simulink model "CRITIS_1_full"  (R2022b)
settings: Solver=VariableStepAuto  StartTime=0.0  StopTime=7  RelTol=1e-3
(part 6 of 13)

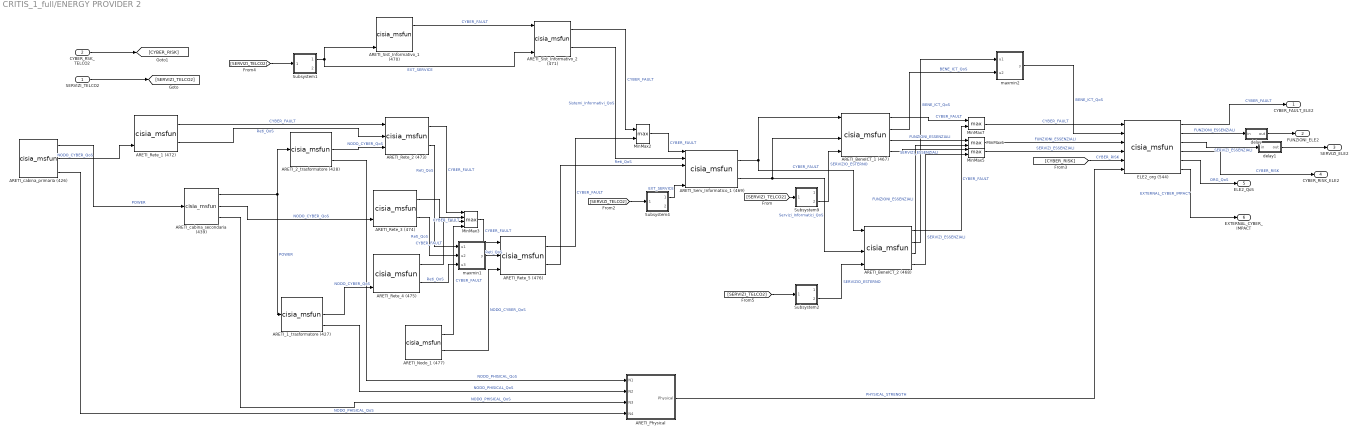
== system CRITIS_1_full/ENERGY PROVIDER 2 ==
  SERVIZI_TELCO2 : Inport
  CYBER_RSK_TELCO2 : Inport  Port=2
  ARETI_1_trasformatore (427) : M-S-Function  FunctionName=cisia_msfun  Parameters=Parameter1, Parameter2, Parameter3, resources, Parameter10, codeupdate, step_received, step_computed, dynamic_computed, step_sended, id_entity, id_project, id_type, name_type, color  mask(S-function:msfcn_unit_delay){Parameter1='ARETI_1_trasformatore', Parameter2=1, Parameter3='Iside', resources=|, Parameter10=off, codeupdate=off, step_received=|, step_computed=, dynamic_computed=, step_sended=|, id_entity=427, id_project=14, id_type=105, name_type=Nodo_Trasformatore, color=#DCF6F7}
      mask resources=|
      | *** INPUT RESOURCES ***
      | NUM_INPUTS 1
      | POWER (1)
      |
      | *** STATE VARIABLES ***
      | NUM_VARIABLES 8
      | Operative_Level(NUMERIC)(1)(1)
      | Mechanical_Fault(NUMERIC)(1)(0)
      | Power_Fault(NUMERIC)(1)(0)
      | Fire_Fault(NUMERIC)(1)(0)
      | Physical_Fault(NUMERIC)(1)(0)
      | Op_Level2(NUMERIC_ARRAY)(2)(0  0)
      | Possibility_Value(NUMERIC)(1)(0)
      | Necessity_Value(NUMERIC)(1)(0)
      |
      | *** OUTPUT RESOURCES ***
      | NUM_OUTPUTS 3
      | POWER_QoS (1)
      | NODO_CYBER_QoS (2)
      | NODO_PHISICAL_QoS (1)
      mask step_received=|
      | Power_Fault = 1-POWER;
      |
      | Physical_Fault = max([Mechanical_Fault Fire_Fault]);
      |
      | Operative_Level = (1-Power_Fault)*(1-Physical_Fault);
      |
      | % Il primo elemento rappersenta possibility e si combima
      | % con il max in quanto rende conto del caso migliore
      | % (perche OL)
      |
      | Op_Level2(1)=  min([1-Power_Fault 1-Physical_Fault]);
      |
      | % Il secondo elemento rappersenta necessity e si combima
      | % con il min in quanto rende conto del caso peggiore
      | % (perche OL)
      |
      | Op_Level2(2)= min([1-Power_Fault 1-Physical_Fault]);
      |
      | Possibility_Value = Op_Level2(1);
      | Necessity_Value = Op_Level2(2);
      mask step_sended=|
      | POWER_QoS = 1-Power_Fault;
      |
      | NODO_CYBER_QoS=Op_Level2;
      |
      | NODO_PHISICAL_QoS=1-Physical_Fault;
      mask prompts: Parameter1 "entity name"; Parameter2 "sampling time"; Parameter3 "project"; resources "input resources and state variables"; Parameter10 "Bring state variables to output"; codeupdate "update code from mask"
      mask help: This is a level-2 MATLAB file S-function which demonstrates CISIA entity
      mask DialogControl Container1 Prompt: All parameters
      mask Display: disp('Nodo_Trasformatore')
  ARETI_2_trasformatore (428) : M-S-Function  FunctionName=cisia_msfun  Parameters=Parameter1, Parameter2, Parameter3, resources, Parameter10, codeupdate, step_received, step_computed, dynamic_computed, step_sended, id_entity, id_project, id_type, name_type, color  mask(S-function:msfcn_unit_delay){Parameter1='ARETI_2_trasformatore', Parameter2=1, Parameter3='Iside', resources=|, Parameter10=off, codeupdate=off, step_received=|, step_computed=, dynamic_computed=, step_sended=|, id_entity=428, id_project=14, id_type=105, name_type=Nodo_Trasformatore, color=#DCF6F7}
      mask resources=|
      | *** INPUT RESOURCES ***
      | NUM_INPUTS 1
      | POWER (1)
      |
      | *** STATE VARIABLES ***
      | NUM_VARIABLES 8
      | Operative_Level(NUMERIC)(1)(1)
      | Mechanical_Fault(NUMERIC)(1)(0)
      | Power_Fault(NUMERIC)(1)(0)
      | Fire_Fault(NUMERIC)(1)(0)
      | Physical_Fault(NUMERIC)(1)(0)
      | Op_Level2(NUMERIC_ARRAY)(2)(0  0)
      | Possibility_Value(NUMERIC)(1)(0)
      | Necessity_Value(NUMERIC)(1)(0)
      |
      | *** OUTPUT RESOURCES ***
      | NUM_OUTPUTS 3
      | POWER_QoS (1)
      | NODO_CYBER_QoS (2)
      | NODO_PHISICAL_QoS (1)
      mask step_received=|
      | Power_Fault = 1-POWER;
      |
      | Physical_Fault = max([Mechanical_Fault Fire_Fault]);
      |
      | Operative_Level = (1-Power_Fault)*(1-Physical_Fault);
      |
      | % Il primo elemento rappersenta possibility e si combima
      | % con il max in quanto rende conto del caso migliore
      | % (perche OL)
      |
      | Op_Level2(1)=  min([1-Power_Fault 1-Physical_Fault]);
      |
      | % Il secondo elemento rappersenta necessity e si combima
      | % con il min in quanto rende conto del caso peggiore
      | % (perche OL)
      |
      | Op_Level2(2)= min([1-Power_Fault 1-Physical_Fault]);
      |
      | Possibility_Value = Op_Level2(1);
      | Necessity_Value = Op_Level2(2);
      mask step_sended=|
      | POWER_QoS = 1-Power_Fault;
      |
      | NODO_CYBER_QoS=Op_Level2;
      |
      | NODO_PHISICAL_QoS=1-Physical_Fault;
      mask prompts: Parameter1 "entity name"; Parameter2 "sampling time"; Parameter3 "project"; resources "input resources and state variables"; Parameter10 "Bring state variables to output"; codeupdate "update code from mask"
      mask help: This is a level-2 MATLAB file S-function which demonstrates CISIA entity
      mask DialogControl Container1 Prompt: All parameters
      mask Display: disp('Nodo_Trasformatore')
  ARETI_BeneICT_1 (467) : M-S-Function  FunctionName=cisia_msfun  Parameters=Parameter1, Parameter2, Parameter3, resources, Parameter10, codeupdate, step_received, step_computed, dynamic_computed, step_sended, id_entity, id_project, id_type, name_type, color  mask(S-function:msfcn_unit_delay){Parameter1='ARETI_BeneICT_1', Parameter2=1, Parameter3='Iside', resources=|, Parameter10=off, codeupdate=off, step_received=|, step_computed=, dynamic_computed=, step_sended=|, id_entity=467, id_project=14, id_type=108, name_type=BeneICT, color=#64D413}
      mask resources=|
      | *** INPUT RESOURCES ***
      | NUM_INPUTS 6
      | CYBER_FAULT (25)
      | Sistemi_Informativi_QoS (2)
      | Reti_QoS (2)
      | Servizi_Informatici_QoS (2)
      | BENE_ICT_QoS (2)
      | SERVIZIO_ESTERNO (20)
      |
      | *** STATE VARIABLES ***
      | NUM_VARIABLES 34
      | Operative_Level(NUMERIC)(1)(1)
      | Dos_attack(NUMERIC)(1)(0)
      | MITM_attack(NUMERIC)(1)(0)
      | Virus_Attack(NUMERIC)(1)(0)
      | Port_Scan_Attack(NUMERIC)(1)(0)
      | Cyber_Fault(NUMERIC_ARRAY)(25)(0  0  0  0  0  0  0  0  0  0  0  0  0  0  0  0  0  0  0  0  0  0  0  0  0)
      | BGP_hijacking(NUMERIC)(1)(0)
      | Unauthorized_Access(NUMERIC)(1)(0)
      | Consumed_Services(NUMERIC_ARRAY)(10)(0  0  0  0  0  0  0  0  0  0)
      | Service_Fault(NUMERIC)(1)(0)
      | BotNet_Attack(NUMERIC)(1)(0)
      | Data_Corruption(NUMERIC)(1)(0)
      | Rouge_Access(NUMERIC)(1)(0)
      | syslog_adm_login(NUMERIC)(1)(0)
      | SW_Change(NUMERIC)(1)(0)
      | Config_Change(NUMERIC)(1)(0)
      | Port_Saturation(NUMERIC)(1)(0)
      | Congestion_Fault(NUMERIC)(1)(0)
      | Route_Poisoning(NUMERIC)(1)(0)
      | Interface_Down(NUMERIC)(1)(0)
      | Port_Isolation(NUMERIC)(1)(0)
      | Unknown_Device(NUMERIC)(1)(0)
      | USB_Device_Insertion(NUMERIC)(1)(0)
      | SW_Fault(NUMERIC)(1)(0)
      | Servizi_Essenziali(NUMERIC_ARRAY)(10)(1  0  0  0  0  0  0  0  0  0)
      | Funzioni_Essenziali(NUMERIC_ARRAY)(10)(0  0  0  0  0  0  0  0  0  0)
      | Consumed_Functions(NUMERIC_ARRAY)(10)(0  0  0  0  0  0  0  0  0  0)
      | Internal_Cyber_Risk(NUMERIC)(1)(0)
      | Data_Breach(NUMERIC)(1)(0)
      | availability_fault(NUMERIC)(1)(0)
      | Ransomware(NUMERIC)(1)(0)
      | Op_Level2(NUMERIC_ARRAY)(2)(0  0)
      | Possibility_Value(NUMERIC)(1)(0)
      | Necessity_Value(NUMERIC)(1)(0)
      |
      | *** OUTPUT RESOURCES ***
      | NUM_OUTPUTS 4
      | CYBER_FAULT (25)
      | BENE_ICT_QoS (2)
      | FUNZIONI_ESSENZIALI (10)
      | SERVIZI_ESSENZIALI (10)
      mask step_received=|
      | cyber_event=zeros(1,25);
      | cyber_event(1)=Dos_attack;
      | cyber_event(2)=MITM_attack;
      | cyber_event(3)=Virus_Attack;
      | cyber_event(4)=Port_Scan_Attack;
      | cyber_event(5)=BGP_hijacking;
      | cyber_event(6)=BotNet_Attack;
      | cyber_event(7)=Data_Corruption;
      | cyber_event(8)=SW_Change;
      | cyber_event(9)=Config_Change;
      | cyber_event(10)=Port_Saturation;
      | cyber_event(11)=Data_Breach;
      | cyber_event(12)=Unauthorized_Access;
      | cyber_event(13)=Unknown_Device;
      | cyber_event(14)=Congestion_Fault;
      | cyber_event(15)=Interface_Down;
      | cyber_event(16)=Port_Isolation;
      | cyber_event(17)=Rouge_Access;
      | cyber_event(18)=Route_Poisoning;
      | cyber_event(19)=SW_Fault;
      | cyber_event(20)=syslog_adm_login;
      | cyber_event(21)=USB_Device_Insertion;
      | cyber_event(22)=Ransomware;
      | cyber_event(23)=0;
      | cyber_event(24)=0;
      | cyber_event(25)=0;
      |
      | Cyber_Fault=max(CYBER_FAULT, transpose(cyber_event));
      |
      | Consumed_Services=SERVIZIO_ESTERNO(1:10);
      | Consumed_Functions=SERVIZIO_ESTERNO(11:20);
      |
      | Service_Fault=max(abs(Servizi_Essenziali-Consumed_Services));
      |
      | availability_fault=1-min([(1-0.5*max(Cyber_Fault)) min(Reti_QoS) min(Sistemi_Informativi_QoS) min(Servizi_Informatici_QoS) min(BENE_ICT_QoS)]);
      |
      | Operative_Level=min([(1-0.5*max(Cyber_Fault)) mean(Reti_QoS) mean(Sistemi_Informativi_QoS) mean(Servizi_Informatici_QoS) mean(BENE_ICT_QoS) 1-Service_Fault]);
      |
      | % Il primo elemento rappersenta possibility e si combima
      | % con il max in quanto rende conto del caso migliore
      | % (perche OL)
      |
      | BNICT=BENE_ICT_QoS;
      |
      | Op_Level2(1)=  min([1-0.3*max(Cyber_Fault) max([use_elem(Reti_QoS,1) use_elem(Sistemi_Informativi_QoS,1) use_elem(Servizi_Informatici_QoS,1) use_elem(BENE_ICT_QoS,1)]) 1-Service_Fault]);
      |
      | % Il secondo elemento rappresenta necessity e si combima
      | % con il min in quanto rende conto del caso peggiore
      | % (perche OL)
      |
      |
      |
      | Op_Level2(2)= min([1-0.6*max(Cyber_Fault) min([use_elem(Reti_QoS,2) use_elem(Sistemi_Informativi_QoS,2) use_elem(Servizi_Informatici_QoS,2) use_elem(BENE_ICT_QoS,2)]) 1-Service_Fault]);
      |
      | Possibility_Value = Op_Level2(1);
      | Necessity_Value = Op_Level2(2);
      mask step_sended=|
      | CYBER_FAULT=Cyber_Fault;
      |
      | FUNZIONI_ESSENZIALI=(1-availability_fault)*Funzioni_Essenziali.*Consumed_Functions;
      |
      | SERVIZI_ESSENZIALI=(1-availability_fault)*Servizi_Essenziali.*Consumed_Services;
      |
      | BENE_ICT_QoS=Op_Level2;
      mask prompts: Parameter1 "entity name"; Parameter2 "sampling time"; Parameter3 "project"; resources "input resources and state variables"; Parameter10 "Bring state variables to output"; codeupdate "update code from mask"
      mask help: This is a level-2 MATLAB file S-function which demonstrates CISIA entity
      mask DialogControl Container1 Prompt: All parameters
      mask Display: disp('BeneICT');port_label('input',2,'\color{yellow}\spadesuit','texmode','on');port_label('input',3,'\color{yellow}\spadesuit','texmode','on');port_label('input',5,'\color{yellow}\spadesuit','texmode','on')
  ARETI_BeneICT_2 (468) : M-S-Function  FunctionName=cisia_msfun  Parameters=Parameter1, Parameter2, Parameter3, resources, Parameter10, codeupdate, step_received, step_computed, dynamic_computed, step_sended, id_entity, id_project, id_type, name_type, color  mask(S-function:msfcn_unit_delay){Parameter1='ARETI_BeneICT_2', Parameter2=1, Parameter3='Iside', resources=|, Parameter10=off, codeupdate=off, step_received=|, step_computed=, dynamic_computed=, step_sended=|, id_entity=468, id_project=14, id_type=108, name_type=BeneICT, color=#64D413}
      mask resources=|
      | *** INPUT RESOURCES ***
      | NUM_INPUTS 6
      | CYBER_FAULT (25)
      | Sistemi_Informativi_QoS (2)
      | Reti_QoS (2)
      | Servizi_Informatici_QoS (2)
      | BENE_ICT_QoS (2)
      | SERVIZIO_ESTERNO (20)
      |
      | *** STATE VARIABLES ***
      | NUM_VARIABLES 34
      | Operative_Level(NUMERIC)(1)(1)
      | Dos_attack(NUMERIC)(1)(0)
      | MITM_attack(NUMERIC)(1)(0)
      | Virus_Attack(NUMERIC)(1)(0)
      | Port_Scan_Attack(NUMERIC)(1)(0)
      | Cyber_Fault(NUMERIC_ARRAY)(25)(0  0  0  0  0  0  0  0  0  0  0  0  0  0  0  0  0  0  0  0  0  0  0  0  0)
      | BGP_hijacking(NUMERIC)(1)(0)
      | Unauthorized_Access(NUMERIC)(1)(0)
      | Consumed_Services(NUMERIC_ARRAY)(10)(0  0  0  0  0  0  0  0  0  0)
      | Service_Fault(NUMERIC)(1)(0)
      | BotNet_Attack(NUMERIC)(1)(0)
      | Data_Corruption(NUMERIC)(1)(0)
      | Rouge_Access(NUMERIC)(1)(0)
      | syslog_adm_login(NUMERIC)(1)(0)
      | SW_Change(NUMERIC)(1)(0)
      | Config_Change(NUMERIC)(1)(0)
      | Port_Saturation(NUMERIC)(1)(0)
      | Congestion_Fault(NUMERIC)(1)(0)
      | Route_Poisoning(NUMERIC)(1)(0)
      | Interface_Down(NUMERIC)(1)(0)
      | Port_Isolation(NUMERIC)(1)(0)
      | Unknown_Device(NUMERIC)(1)(0)
      | USB_Device_Insertion(NUMERIC)(1)(0)
      | SW_Fault(NUMERIC)(1)(0)
      | Servizi_Essenziali(NUMERIC_ARRAY)(10)(0  1  0  0  0  0  0  0  0  0)
      | Funzioni_Essenziali(NUMERIC_ARRAY)(10)(0  0  0  0  0  0  0  0  0  0)
      | Consumed_Functions(NUMERIC_ARRAY)(10)(0  0  0  0  0  0  0  0  0  0)
      | Internal_Cyber_Risk(NUMERIC)(1)(0)
      | Data_Breach(NUMERIC)(1)(0)
      | availability_fault(NUMERIC)(1)(0)
      | Ransomware(NUMERIC)(1)(0)
      | Op_Level2(NUMERIC_ARRAY)(2)(0  0)
      | Possibility_Value(NUMERIC)(1)(0)
      | Necessity_Value(NUMERIC)(1)(0)
      |
      | *** OUTPUT RESOURCES ***
      | NUM_OUTPUTS 4
      | CYBER_FAULT (25)
      | BENE_ICT_QoS (2)
      | FUNZIONI_ESSENZIALI (10)
      | SERVIZI_ESSENZIALI (10)
      mask step_received=|
      | cyber_event=zeros(1,25);
      | cyber_event(1)=Dos_attack;
      | cyber_event(2)=MITM_attack;
      | cyber_event(3)=Virus_Attack;
      | cyber_event(4)=Port_Scan_Attack;
      | cyber_event(5)=BGP_hijacking;
      | cyber_event(6)=BotNet_Attack;
      | cyber_event(7)=Data_Corruption;
      | cyber_event(8)=SW_Change;
      | cyber_event(9)=Config_Change;
      | cyber_event(10)=Port_Saturation;
      | cyber_event(11)=Data_Breach;
      | cyber_event(12)=Unauthorized_Access;
      | cyber_event(13)=Unknown_Device;
      | cyber_event(14)=Congestion_Fault;
      | cyber_event(15)=Interface_Down;
      | cyber_event(16)=Port_Isolation;
      | cyber_event(17)=Rouge_Access;
      | cyber_event(18)=Route_Poisoning;
      | cyber_event(19)=SW_Fault;
      | cyber_event(20)=syslog_adm_login;
      | cyber_event(21)=USB_Device_Insertion;
      | cyber_event(22)=Ransomware;
      | cyber_event(23)=0;
      | cyber_event(24)=0;
      | cyber_event(25)=0;
      |
      | Cyber_Fault=max(CYBER_FAULT, transpose(cyber_event));
      |
      | Consumed_Services=SERVIZIO_ESTERNO(1:10);
      | Consumed_Functions=SERVIZIO_ESTERNO(11:20);
      |
      | Service_Fault=max(abs(Servizi_Essenziali-Consumed_Services));
      |
      | availability_fault=1-min([(1-0.5*max(Cyber_Fault)) min(Reti_QoS) min(Sistemi_Informativi_QoS) min(Servizi_Informatici_QoS) min(BENE_ICT_QoS)]);
      |
      | Operative_Level=min([(1-0.5*max(Cyber_Fault)) mean(Reti_QoS) mean(Sistemi_Informativi_QoS) mean(Servizi_Informatici_QoS) mean(BENE_ICT_QoS) 1-Service_Fault]);
      |
      | % Il primo elemento rappersenta possibility e si combima
      | % con il max in quanto rende conto del caso migliore
      | % (perche OL)
      |
      | BNICT=BENE_ICT_QoS;
      |
      | Op_Level2(1)=  min([1-0.3*max(Cyber_Fault) max([use_elem(Reti_QoS,1) use_elem(Sistemi_Informativi_QoS,1) use_elem(Servizi_Informatici_QoS,1) use_elem(BENE_ICT_QoS,1)]) 1-Service_Fault]);
      |
      | % Il secondo elemento rappresenta necessity e si combima
      | % con il min in quanto rende conto del caso peggiore
      | % (perche OL)
      |
      |
      |
      | Op_Level2(2)= min([1-0.6*max(Cyber_Fault) min([use_elem(Reti_QoS,2) use_elem(Sistemi_Informativi_QoS,2) use_elem(Servizi_Informatici_QoS,2) use_elem(BENE_ICT_QoS,2)]) 1-Service_Fault]);
      |
      | Possibility_Value = Op_Level2(1);
      | Necessity_Value = Op_Level2(2);
      mask step_sended=|
      | CYBER_FAULT=Cyber_Fault;
      |
      | FUNZIONI_ESSENZIALI=(1-availability_fault)*Funzioni_Essenziali.*Consumed_Functions;
      |
      | SERVIZI_ESSENZIALI=(1-availability_fault)*Servizi_Essenziali.*Consumed_Services;
      |
      | BENE_ICT_QoS=Op_Level2;
      mask prompts: Parameter1 "entity name"; Parameter2 "sampling time"; Parameter3 "project"; resources "input resources and state variables"; Parameter10 "Bring state variables to output"; codeupdate "update code from mask"
      mask help: This is a level-2 MATLAB file S-function which demonstrates CISIA entity
      mask DialogControl Container1 Prompt: All parameters
      mask Display: disp('BeneICT');port_label('input',2,'\color{yellow}\spadesuit','texmode','on');port_label('input',3,'\color{yellow}\spadesuit','texmode','on');port_label('input',5,'\color{yellow}\spadesuit','texmode','on')
  ARETI_Nodo_1 (477) : M-S-Function  FunctionName=cisia_msfun  Parameters=Parameter1, Parameter2, Parameter3, resources, Parameter10, codeupdate, step_received, step_computed, dynamic_computed, step_sended, id_entity, id_project, id_type, name_type, color  mask(S-function:msfcn_unit_delay){Parameter1='ARETI_Nodo_1', Parameter2=1, Parameter3='Iside', resources=|, Parameter10=off, codeupdate=off, step_received=|, step_computed=, dynamic_computed=, step_sended=|, id_entity=477, id_project=14, id_type=109, name_type=Nodo_Datacenter, color=#DCF6F7}
      mask resources=|
      | *** INPUT RESOURCES ***
      | NUM_INPUTS 0
      |
      | *** STATE VARIABLES ***
      | NUM_VARIABLES 32
      | Operative_Level(NUMERIC)(1)(1)
      | Dos_attack(NUMERIC)(1)(0)
      | MITM_attack(NUMERIC)(1)(0)
      | Virus_Attack(NUMERIC)(1)(0)
      | Port_Scan_Attack(NUMERIC)(1)(0)
      | Cyber_Fault(NUMERIC_ARRAY)(25)(0  0  0  0  0  0  0  0  0  0  0  0  0  0  0  0  0  0  0  0  0  0  0  0  0)
      | BGP_hijacking(NUMERIC)(1)(0)
      | Mechanical_Fault(NUMERIC)(1)(0)
      | Unauthorized_Access(NUMERIC)(1)(0)
      | Conn_Fault(NUMERIC)(1)(0)
      | BotNet_Attack(NUMERIC)(1)(0)
      | Data_Corruption(NUMERIC)(1)(0)
      | Rouge_Access(NUMERIC)(1)(0)
      | syslog_adm_login(NUMERIC)(1)(0)
      | SW_Change(NUMERIC)(1)(0)
      | Config_Change(NUMERIC)(1)(0)
      | Port_Saturation(NUMERIC)(1)(0)
      | Congestion_Fault(NUMERIC)(1)(0)
      | Route2(NUMERIC)(1)(0)
      | Route_Poisoning(NUMERIC)(1)(0)
      | Interface_Down(NUMERIC)(1)(0)
      | Port_Isolation(NUMERIC)(1)(0)
      | Unknown_Device(NUMERIC)(1)(0)
      | USB_Device_Insertion(NUMERIC)(1)(0)
      | GEO_localization(STRING)(100)()
      | SW_Fault(NUMERIC)(1)(0)
      | Internal_Cyber_Risk(NUMERIC)(1)(0)
      | Data_Breach(NUMERIC)(1)(0)
      | Ransomware(NUMERIC)(1)(0)
      | Op_Level2(NUMERIC_ARRAY)(2)(0  0)
      | Possibility_Value(NUMERIC)(1)(0)
      | Necessity_Value(NUMERIC)(1)(0)
      |
      | *** OUTPUT RESOURCES ***
      | NUM_OUTPUTS 2
      | CYBER_FAULT (25)
      | NODO_CYBER_QoS (2)
      mask step_received=|
      | cyber_event=zeros(1,25);
      | cyber_event(1)=Dos_attack;
      | cyber_event(2)=MITM_attack;
      | cyber_event(3)=Virus_Attack;
      | cyber_event(4)=Port_Scan_Attack;
      | cyber_event(5)=BGP_hijacking;
      | cyber_event(6)=BotNet_Attack;
      | cyber_event(7)=Data_Corruption;
      | cyber_event(8)=SW_Change;
      | cyber_event(9)=Config_Change;
      | cyber_event(10)=Port_Saturation;
      | cyber_event(11)=Data_Breach;
      | cyber_event(12)=Unauthorized_Access;
      | cyber_event(13)=Unknown_Device;
      | cyber_event(14)=Congestion_Fault;
      | cyber_event(15)=Interface_Down;
      | cyber_event(16)=Port_Isolation;
      | cyber_event(17)=Rouge_Access;
      | cyber_event(18)=Route_Poisoning;
      | cyber_event(19)=SW_Fault;
      | cyber_event(20)=syslog_adm_login;
      | cyber_event(21)=USB_Device_Insertion;
      | cyber_event(22)=Ransomware;
      | cyber_event(23)=0;
      | cyber_event(24)=0;
      | cyber_event(25)=0;
      |
      | Cyber_Fault=transpose(cyber_event);
      |
      | Conn_Fault=max([Dos_attack BGP_hijacking Route_Poisoning Interface_Down Mechanical_Fault] );
      |
      |
      | Operative_Level=min((1-Conn_Fault),(1-0.5*max(Cyber_Fault)));
      |
      | % Il primo elemento rappersenta possibility e si combima
      | % con il max in quanto rende conto del caso migliore
      | % (perche OL)
      |
      | Op_Level2(1)=  min([1-0.3*max(Cyber_Fault) 1-Conn_Fault]);
      |
      | % Il secondo elemento rappersenta necessity e si combima
      | % con il min in quanto rende conto del caso peggiore
      | % (perche OL)
      |
      | Op_Level2(2)= min([1-0.6*max(Cyber_Fault) 1-Conn_Fault]);
      |
      | Possibility_Value = Op_Level2(1);
      | Necessity_Value = Op_Level2(2);
      mask step_sended=|
      | CYBER_FAULT=Cyber_Fault;
      |
      |
      | NODO_CYBER_QoS=Op_Level2;
      mask prompts: Parameter1 "entity name"; Parameter2 "sampling time"; Parameter3 "project"; resources "input resources and state variables"; Parameter10 "Bring state variables to output"; codeupdate "update code from mask"
      mask help: This is a level-2 MATLAB file S-function which demonstrates CISIA entity
      mask DialogControl Container1 Prompt: All parameters
      mask Display: disp('Nodo_Datacenter')
  ARETI_Physical : MATLAB Function  TreatAsAtomicUnit=on
  ARETI_Rete_1 (472) : M-S-Function  FunctionName=cisia_msfun  Parameters=Parameter1, Parameter2, Parameter3, resources, Parameter10, codeupdate, step_received, step_computed, dynamic_computed, step_sended, id_entity, id_project, id_type, name_type, color  mask(S-function:msfcn_unit_delay){Parameter1='ARETI_Rete_1', Parameter2=1, Parameter3='Iside', resources=|, Parameter10=off, codeupdate=off, step_received=|, step_computed=, dynamic_computed=, step_sended=|, id_entity=472, id_project=14, id_type=82, name_type=Reti_Sito, color=#45B5ED}
      mask resources=|
      | *** INPUT RESOURCES ***
      | NUM_INPUTS 3
      | CYBER_FAULT (25)
      | Reti_QoS (2)
      | NODO_CYBER_QoS (2)
      |
      | *** STATE VARIABLES ***
      | NUM_VARIABLES 34
      | Operative_Level(NUMERIC)(1)(1)
      | Dos_attack(NUMERIC)(1)(0)
      | MITM_attack(NUMERIC)(1)(0)
      | Virus_Attack(NUMERIC)(1)(0)
      | Port_Scan_Attack(NUMERIC)(1)(0)
      | Cyber_Fault(NUMERIC_ARRAY)(25)(0  0  0  0  0  0  0  0  0  0  0  0  0  0  0  0  0  0  0  0  0  0  0  0  0)
      | BGP_hijacking(NUMERIC)(1)(0)
      | Mechanical_Fault(NUMERIC)(1)(0)
      | Unauthorized_Access(NUMERIC)(1)(0)
      | Conn_Fault(NUMERIC)(1)(0)
      | BotNet_Attack(NUMERIC)(1)(0)
      | Data_Corruption(NUMERIC)(1)(0)
      | Rouge_Access(NUMERIC)(1)(0)
      | syslog_adm_login(NUMERIC)(1)(0)
      | SW_Change(NUMERIC)(1)(0)
      | Config_Change(NUMERIC)(1)(0)
      | Port_Saturation(NUMERIC)(1)(0)
      | Congestion_Fault(NUMERIC)(1)(0)
      | Physical_Fault(NUMERIC)(1)(0)
      | Route2(NUMERIC)(1)(0)
      | Route_Poisoning(NUMERIC)(1)(0)
      | Interface_Down(NUMERIC)(1)(0)
      | Port_Isolation(NUMERIC)(1)(0)
      | Unknown_Device(NUMERIC)(1)(0)
      | USB_Device_Insertion(NUMERIC)(1)(0)
      | Risorsa(NUMERIC)(1)(0)
      | GEO_localization(STRING)(100)()
      | SW_Fault(NUMERIC)(1)(0)
      | Internal_Cyber_Risk(NUMERIC)(1)(0)
      | Data_Breach(NUMERIC)(1)(0)
      | Ransomware(NUMERIC)(1)(0)
      | Op_Level2(NUMERIC_ARRAY)(2)(0  0)
      | Possibility_Value(NUMERIC)(1)(0)
      | Necessity_Value(NUMERIC)(1)(0)
      |
      | *** OUTPUT RESOURCES ***
      | NUM_OUTPUTS 2
      | CYBER_FAULT (25)
      | Reti_QoS (2)
      mask step_received=|
      | cyber_event=zeros(1,25);
      | cyber_event(1)=Dos_attack;
      | cyber_event(2)=MITM_attack;
      | cyber_event(3)=Virus_Attack;
      | cyber_event(4)=Port_Scan_Attack;
      | cyber_event(5)=BGP_hijacking;
      | cyber_event(6)=BotNet_Attack;
      | cyber_event(7)=Data_Corruption;
      | cyber_event(8)=SW_Change;
      | cyber_event(9)=Config_Change;
      | cyber_event(10)=Port_Saturation;
      | cyber_event(11)=Data_Breach;
      | cyber_event(12)=Unauthorized_Access;
      | cyber_event(13)=Unknown_Device;
      | cyber_event(14)=Congestion_Fault;
      | cyber_event(15)=Interface_Down;
      | cyber_event(16)=Port_Isolation;
      | cyber_event(17)=Rouge_Access;
      | cyber_event(18)=Route_Poisoning;
      | cyber_event(19)=SW_Fault;
      | cyber_event(20)=syslog_adm_login;
      | cyber_event(21)=USB_Device_Insertion;
      | cyber_event(22)=Ransomware;
      | cyber_event(23)=0;
      | cyber_event(24)=0;
      | cyber_event(25)=0;
      |
      | Cyber_Fault=max(CYBER_FAULT, transpose(cyber_event));
      |
      | Conn_Fault=max([Dos_attack BGP_hijacking Route_Poisoning Interface_Down Mechanical_Fault] );
      |
      | Operative_Level=min([(1-Conn_Fault) (1-0.5*max(Cyber_Fault))  mean(Reti_QoS)  mean(NODO_CYBER_QoS)]);
      |
      | % Il primo elemento rappersenta possibility e si combima
      | % con il max in quanto rende conto del caso migliore
      | % (perche OL)
      |
      | Op_Level2(1)=  min([1-0.3*max(Cyber_Fault) max([use_elem(Reti_QoS,1) use_elem(NODO_CYBER_QoS,1)]) 1-Conn_Fault]);
      |
      | % Il secondo elemento rappersenta necessity e si combima
      | % con il min in quanto rende conto del caso peggiore
      | % (perche OL)
      |
      | Op_Level2(2)= min([1-0.6*max(Cyber_Fault) min([use_elem(Reti_QoS,2) use_elem(NODO_CYBER_QoS,2)]) 1-Conn_Fault]);
      |
      | Possibility_Value = Op_Level2(1);
      | Necessity_Value = Op_Level2(2);
      mask step_sended=|
      | CYBER_FAULT=Cyber_Fault;
      |
      |
      | Reti_QoS=Op_Level2;
      mask prompts: Parameter1 "entity name"; Parameter2 "sampling time"; Parameter3 "project"; resources "input resources and state variables"; Parameter10 "Bring state variables to output"; codeupdate "update code from mask"
      mask help: This is a level-2 MATLAB file S-function which demonstrates CISIA entity
      mask DialogControl Container1 Prompt: All parameters
      mask Display: disp('Reti_Sito');port_label('input',1,'\color{yellow}\spadesuit','texmode','on');port_label('input',2,'\color{yellow}\spadesuit','texmode','on')
  ARETI_Rete_2 (473) : M-S-Function  FunctionName=cisia_msfun  Parameters=Parameter1, Parameter2, Parameter3, resources, Parameter10, codeupdate, step_received, step_computed, dynamic_computed, step_sended, id_entity, id_project, id_type, name_type, color  mask(S-function:msfcn_unit_delay){Parameter1='ARETI_Rete_2', Parameter2=1, Parameter3='Iside', resources=|, Parameter10=off, codeupdate=off, step_received=|, step_computed=, dynamic_computed=, step_sended=|, id_entity=473, id_project=14, id_type=82, name_type=Reti_Sito, color=#45B5ED}
      mask resources=|
      | *** INPUT RESOURCES ***
      | NUM_INPUTS 3
      | CYBER_FAULT (25)
      | Reti_QoS (2)
      | NODO_CYBER_QoS (2)
      |
      | *** STATE VARIABLES ***
      | NUM_VARIABLES 34
      | Operative_Level(NUMERIC)(1)(1)
      | Dos_attack(NUMERIC)(1)(0)
      | MITM_attack(NUMERIC)(1)(0)
      | Virus_Attack(NUMERIC)(1)(0)
      | Port_Scan_Attack(NUMERIC)(1)(0)
      | Cyber_Fault(NUMERIC_ARRAY)(25)(0  0  0  0  0  0  0  0  0  0  0  0  0  0  0  0  0  0  0  0  0  0  0  0  0)
      | BGP_hijacking(NUMERIC)(1)(0)
      | Mechanical_Fault(NUMERIC)(1)(0)
      | Unauthorized_Access(NUMERIC)(1)(0)
      | Conn_Fault(NUMERIC)(1)(0)
      | BotNet_Attack(NUMERIC)(1)(0)
      | Data_Corruption(NUMERIC)(1)(0)
      | Rouge_Access(NUMERIC)(1)(0)
      | syslog_adm_login(NUMERIC)(1)(0)
      | SW_Change(NUMERIC)(1)(0)
      | Config_Change(NUMERIC)(1)(0)
      | Port_Saturation(NUMERIC)(1)(0)
      | Congestion_Fault(NUMERIC)(1)(0)
      | Physical_Fault(NUMERIC)(1)(0)
      | Route2(NUMERIC)(1)(0)
      | Route_Poisoning(NUMERIC)(1)(0)
      | Interface_Down(NUMERIC)(1)(0)
      | Port_Isolation(NUMERIC)(1)(0)
      | Unknown_Device(NUMERIC)(1)(0)
      | USB_Device_Insertion(NUMERIC)(1)(0)
      | Risorsa(NUMERIC)(1)(0)
      | GEO_localization(STRING)(100)()
      | SW_Fault(NUMERIC)(1)(0)
      | Internal_Cyber_Risk(NUMERIC)(1)(0)
      | Data_Breach(NUMERIC)(1)(0)
      | Ransomware(NUMERIC)(1)(0)
      | Op_Level2(NUMERIC_ARRAY)(2)(0  0)
      | Possibility_Value(NUMERIC)(1)(0)
      | Necessity_Value(NUMERIC)(1)(0)
      |
      | *** OUTPUT RESOURCES ***
      | NUM_OUTPUTS 2
      | CYBER_FAULT (25)
      | Reti_QoS (2)
      mask step_received=|
      | cyber_event=zeros(1,25);
      | cyber_event(1)=Dos_attack;
      | cyber_event(2)=MITM_attack;
      | cyber_event(3)=Virus_Attack;
      | cyber_event(4)=Port_Scan_Attack;
      | cyber_event(5)=BGP_hijacking;
      | cyber_event(6)=BotNet_Attack;
      | cyber_event(7)=Data_Corruption;
      | cyber_event(8)=SW_Change;
      | cyber_event(9)=Config_Change;
      | cyber_event(10)=Port_Saturation;
      | cyber_event(11)=Data_Breach;
      | cyber_event(12)=Unauthorized_Access;
      | cyber_event(13)=Unknown_Device;
      | cyber_event(14)=Congestion_Fault;
      | cyber_event(15)=Interface_Down;
      | cyber_event(16)=Port_Isolation;
      | cyber_event(17)=Rouge_Access;
      | cyber_event(18)=Route_Poisoning;
      | cyber_event(19)=SW_Fault;
      | cyber_event(20)=syslog_adm_login;
      | cyber_event(21)=USB_Device_Insertion;
      | cyber_event(22)=Ransomware;
      | cyber_event(23)=0;
      | cyber_event(24)=0;
      | cyber_event(25)=0;
      |
      | Cyber_Fault=max(CYBER_FAULT, transpose(cyber_event));
      |
      | Conn_Fault=max([Dos_attack BGP_hijacking Route_Poisoning Interface_Down Mechanical_Fault] );
      |
      | Operative_Level=min([(1-Conn_Fault) (1-0.5*max(Cyber_Fault))  mean(Reti_QoS)  mean(NODO_CYBER_QoS)]);
      |
      | % Il primo elemento rappersenta possibility e si combima
      | % con il max in quanto rende conto del caso migliore
      | % (perche OL)
      |
      | Op_Level2(1)=  min([1-0.3*max(Cyber_Fault) max([use_elem(Reti_QoS,1) use_elem(NODO_CYBER_QoS,1)]) 1-Conn_Fault]);
      |
      | % Il secondo elemento rappersenta necessity e si combima
      | % con il min in quanto rende conto del caso peggiore
      | % (perche OL)
      |
      | Op_Level2(2)= min([1-0.6*max(Cyber_Fault) min([use_elem(Reti_QoS,2) use_elem(NODO_CYBER_QoS,2)]) 1-Conn_Fault]);
      |
      | Possibility_Value = Op_Level2(1);
      | Necessity_Value = Op_Level2(2);
      mask step_sended=|
      | CYBER_FAULT=Cyber_Fault;
      |
      |
      | Reti_QoS=Op_Level2;
      mask prompts: Parameter1 "entity name"; Parameter2 "sampling time"; Parameter3 "project"; resources "input resources and state variables"; Parameter10 "Bring state variables to output"; codeupdate "update code from mask"
      mask help: This is a level-2 MATLAB file S-function which demonstrates CISIA entity
      mask DialogControl Container1 Prompt: All parameters
      mask Display: disp('Reti_Sito')
  ARETI_Rete_3 (474) : M-S-Function  FunctionName=cisia_msfun  Parameters=Parameter1, Parameter2, Parameter3, resources, Parameter10, codeupdate, step_received, step_computed, dynamic_computed, step_sended, id_entity, id_project, id_type, name_type, color  mask(S-function:msfcn_unit_delay){Parameter1='ARETI_Rete_3', Parameter2=1, Parameter3='Iside', resources=|, Parameter10=off, codeupdate=off, step_received=|, step_computed=, dynamic_computed=, step_sended=|, id_entity=474, id_project=14, id_type=82, name_type=Reti_Sito, color=#45B5ED}
      mask resources=|
      | *** INPUT RESOURCES ***
      | NUM_INPUTS 3
      | CYBER_FAULT (25)
      | Reti_QoS (2)
      | NODO_CYBER_QoS (2)
      |
      | *** STATE VARIABLES ***
      | NUM_VARIABLES 34
      | Operative_Level(NUMERIC)(1)(1)
      | Dos_attack(NUMERIC)(1)(0)
      | MITM_attack(NUMERIC)(1)(0)
      | Virus_Attack(NUMERIC)(1)(0)
      | Port_Scan_Attack(NUMERIC)(1)(0)
      | Cyber_Fault(NUMERIC_ARRAY)(25)(0  0  0  0  0  0  0  0  0  0  0  0  0  0  0  0  0  0  0  0  0  0  0  0  0)
      | BGP_hijacking(NUMERIC)(1)(0)
      | Mechanical_Fault(NUMERIC)(1)(0)
      | Unauthorized_Access(NUMERIC)(1)(0)
      | Conn_Fault(NUMERIC)(1)(0)
      | BotNet_Attack(NUMERIC)(1)(0)
      | Data_Corruption(NUMERIC)(1)(0)
      | Rouge_Access(NUMERIC)(1)(0)
      | syslog_adm_login(NUMERIC)(1)(0)
      | SW_Change(NUMERIC)(1)(0)
      | Config_Change(NUMERIC)(1)(0)
      | Port_Saturation(NUMERIC)(1)(0)
      | Congestion_Fault(NUMERIC)(1)(0)
      | Physical_Fault(NUMERIC)(1)(0)
      | Route2(NUMERIC)(1)(0)
      | Route_Poisoning(NUMERIC)(1)(0)
      | Interface_Down(NUMERIC)(1)(0)
      | Port_Isolation(NUMERIC)(1)(0)
      | Unknown_Device(NUMERIC)(1)(0)
      | USB_Device_Insertion(NUMERIC)(1)(0)
      | Risorsa(NUMERIC)(1)(0)
      | GEO_localization(STRING)(100)()
      | SW_Fault(NUMERIC)(1)(0)
      | Internal_Cyber_Risk(NUMERIC)(1)(0)
      | Data_Breach(NUMERIC)(1)(0)
      | Ransomware(NUMERIC)(1)(0)
      | Op_Level2(NUMERIC_ARRAY)(2)(0  0)
      | Possibility_Value(NUMERIC)(1)(0)
      | Necessity_Value(NUMERIC)(1)(0)
      |
      | *** OUTPUT RESOURCES ***
      | NUM_OUTPUTS 2
      | CYBER_FAULT (25)
      | Reti_QoS (2)
      mask step_received=|
      | cyber_event=zeros(1,25);
      | cyber_event(1)=Dos_attack;
      | cyber_event(2)=MITM_attack;
      | cyber_event(3)=Virus_Attack;
      | cyber_event(4)=Port_Scan_Attack;
      | cyber_event(5)=BGP_hijacking;
      | cyber_event(6)=BotNet_Attack;
      | cyber_event(7)=Data_Corruption;
      | cyber_event(8)=SW_Change;
      | cyber_event(9)=Config_Change;
      | cyber_event(10)=Port_Saturation;
      | cyber_event(11)=Data_Breach;
      | cyber_event(12)=Unauthorized_Access;
      | cyber_event(13)=Unknown_Device;
      | cyber_event(14)=Congestion_Fault;
      | cyber_event(15)=Interface_Down;
      | cyber_event(16)=Port_Isolation;
      | cyber_event(17)=Rouge_Access;
      | cyber_event(18)=Route_Poisoning;
      | cyber_event(19)=SW_Fault;
      | cyber_event(20)=syslog_adm_login;
      | cyber_event(21)=USB_Device_Insertion;
      | cyber_event(22)=Ransomware;
      | cyber_event(23)=0;
      | cyber_event(24)=0;
      | cyber_event(25)=0;
      |
      | Cyber_Fault=max(CYBER_FAULT, transpose(cyber_event));
      |
      | Conn_Fault=max([Dos_attack BGP_hijacking Route_Poisoning Interface_Down Mechanical_Fault] );
      |
      | Operative_Level=min([(1-Conn_Fault) (1-0.5*max(Cyber_Fault))  mean(Reti_QoS)  mean(NODO_CYBER_QoS)]);
      |
      | % Il primo elemento rappersenta possibility e si combima
      | % con il max in quanto rende conto del caso migliore
      | % (perche OL)
      |
      | Op_Level2(1)=  min([1-0.3*max(Cyber_Fault) max([use_elem(Reti_QoS,1) use_elem(NODO_CYBER_QoS,1)]) 1-Conn_Fault]);
      |
      | % Il secondo elemento rappersenta necessity e si combima
      | % con il min in quanto rende conto del caso peggiore
      | % (perche OL)
      |
      | Op_Level2(2)= min([1-0.6*max(Cyber_Fault) min([use_elem(Reti_QoS,2) use_elem(NODO_CYBER_QoS,2)]) 1-Conn_Fault]);
      |
      | Possibility_Value = Op_Level2(1);
      | Necessity_Value = Op_Level2(2);
      mask step_sended=|
      | CYBER_FAULT=Cyber_Fault;
      |
      |
      | Reti_QoS=Op_Level2;
      mask prompts: Parameter1 "entity name"; Parameter2 "sampling time"; Parameter3 "project"; resources "input resources and state variables"; Parameter10 "Bring state variables to output"; codeupdate "update code from mask"
      mask help: This is a level-2 MATLAB file S-function which demonstrates CISIA entity
      mask DialogControl Container1 Prompt: All parameters
      mask Display: disp('Reti_Sito');port_label('input',1,'\color{yellow}\spadesuit','texmode','on');port_label('input',2,'\color{yellow}\spadesuit','texmode','on')
  ARETI_Rete_4 (475) : M-S-Function  FunctionName=cisia_msfun  Parameters=Parameter1, Parameter2, Parameter3, resources, Parameter10, codeupdate, step_received, step_computed, dynamic_computed, step_sended, id_entity, id_project, id_type, name_type, color  mask(S-function:msfcn_unit_delay){Parameter1='ARETI_Rete_4', Parameter2=1, Parameter3='Iside', resources=|, Parameter10=off, codeupdate=off, step_received=|, step_computed=, dynamic_computed=, step_sended=|, id_entity=475, id_project=14, id_type=82, name_type=Reti_Sito, color=#45B5ED}
      mask resources=|
      | *** INPUT RESOURCES ***
      | NUM_INPUTS 3
      | CYBER_FAULT (25)
      | Reti_QoS (2)
      | NODO_CYBER_QoS (2)
      |
      | *** STATE VARIABLES ***
      | NUM_VARIABLES 34
      | Operative_Level(NUMERIC)(1)(1)
      | Dos_attack(NUMERIC)(1)(0)
      | MITM_attack(NUMERIC)(1)(0)
      | Virus_Attack(NUMERIC)(1)(0)
      | Port_Scan_Attack(NUMERIC)(1)(0)
      | Cyber_Fault(NUMERIC_ARRAY)(25)(0  0  0  0  0  0  0  0  0  0  0  0  0  0  0  0  0  0  0  0  0  0  0  0  0)
      | BGP_hijacking(NUMERIC)(1)(0)
      | Mechanical_Fault(NUMERIC)(1)(0)
      | Unauthorized_Access(NUMERIC)(1)(0)
      | Conn_Fault(NUMERIC)(1)(0)
      | BotNet_Attack(NUMERIC)(1)(0)
      | Data_Corruption(NUMERIC)(1)(0)
      | Rouge_Access(NUMERIC)(1)(0)
      | syslog_adm_login(NUMERIC)(1)(0)
      | SW_Change(NUMERIC)(1)(0)
      | Config_Change(NUMERIC)(1)(0)
      | Port_Saturation(NUMERIC)(1)(0)
      | Congestion_Fault(NUMERIC)(1)(0)
      | Physical_Fault(NUMERIC)(1)(0)
      | Route2(NUMERIC)(1)(0)
      | Route_Poisoning(NUMERIC)(1)(0)
      | Interface_Down(NUMERIC)(1)(0)
      | Port_Isolation(NUMERIC)(1)(0)
      | Unknown_Device(NUMERIC)(1)(0)
      | USB_Device_Insertion(NUMERIC)(1)(0)
      | Risorsa(NUMERIC)(1)(0)
      | GEO_localization(STRING)(100)()
      | SW_Fault(NUMERIC)(1)(0)
      | Internal_Cyber_Risk(NUMERIC)(1)(0)
      | Data_Breach(NUMERIC)(1)(0)
      | Ransomware(NUMERIC)(1)(0)
      | Op_Level2(NUMERIC_ARRAY)(2)(0  0)
      | Possibility_Value(NUMERIC)(1)(0)
      | Necessity_Value(NUMERIC)(1)(0)
      |
      | *** OUTPUT RESOURCES ***
      | NUM_OUTPUTS 2
      | CYBER_FAULT (25)
      | Reti_QoS (2)
      mask step_received=|
      | cyber_event=zeros(1,25);
      | cyber_event(1)=Dos_attack;
      | cyber_event(2)=MITM_attack;
      | cyber_event(3)=Virus_Attack;
      | cyber_event(4)=Port_Scan_Attack;
      | cyber_event(5)=BGP_hijacking;
      | cyber_event(6)=BotNet_Attack;
      | cyber_event(7)=Data_Corruption;
      | cyber_event(8)=SW_Change;
      | cyber_event(9)=Config_Change;
      | cyber_event(10)=Port_Saturation;
      | cyber_event(11)=Data_Breach;
      | cyber_event(12)=Unauthorized_Access;
      | cyber_event(13)=Unknown_Device;
      | cyber_event(14)=Congestion_Fault;
      | cyber_event(15)=Interface_Down;
      | cyber_event(16)=Port_Isolation;
      | cyber_event(17)=Rouge_Access;
      | cyber_event(18)=Route_Poisoning;
      | cyber_event(19)=SW_Fault;
      | cyber_event(20)=syslog_adm_login;
      | cyber_event(21)=USB_Device_Insertion;
      | cyber_event(22)=Ransomware;
      | cyber_event(23)=0;
      | cyber_event(24)=0;
      | cyber_event(25)=0;
      |
      | Cyber_Fault=max(CYBER_FAULT, transpose(cyber_event));
      |
      | Conn_Fault=max([Dos_attack BGP_hijacking Route_Poisoning Interface_Down Mechanical_Fault] );
      |
      | Operative_Level=min([(1-Conn_Fault) (1-0.5*max(Cyber_Fault))  mean(Reti_QoS)  mean(NODO_CYBER_QoS)]);
      |
      | % Il primo elemento rappersenta possibility e si combima
      | % con il max in quanto rende conto del caso migliore
      | % (perche OL)
      |
      | Op_Level2(1)=  min([1-0.3*max(Cyber_Fault) max([use_elem(Reti_QoS,1) use_elem(NODO_CYBER_QoS,1)]) 1-Conn_Fault]);
      |
      | % Il secondo elemento rappersenta necessity e si combima
      | % con il min in quanto rende conto del caso peggiore
      | % (perche OL)
      |
      | Op_Level2(2)= min([1-0.6*max(Cyber_Fault) min([use_elem(Reti_QoS,2) use_elem(NODO_CYBER_QoS,2)]) 1-Conn_Fault]);
      |
      | Possibility_Value = Op_Level2(1);
      | Necessity_Value = Op_Level2(2);
      mask step_sended=|
      | CYBER_FAULT=Cyber_Fault;
      |
      |
      | Reti_QoS=Op_Level2;
      mask prompts: Parameter1 "entity name"; Parameter2 "sampling time"; Parameter3 "project"; resources "input resources and state variables"; Parameter10 "Bring state variables to output"; codeupdate "update code from mask"
      mask help: This is a level-2 MATLAB file S-function which demonstrates CISIA entity
      mask DialogControl Container1 Prompt: All parameters
      mask Display: disp('Reti_Sito');port_label('input',1,'\color{yellow}\spadesuit','texmode','on');port_label('input',2,'\color{yellow}\spadesuit','texmode','on')
  ARETI_Rete_5 (476) : M-S-Function  FunctionName=cisia_msfun  Parameters=Parameter1, Parameter2, Parameter3, resources, Parameter10, codeupdate, step_received, step_computed, dynamic_computed, step_sended, id_entity, id_project, id_type, name_type, color  mask(S-function:msfcn_unit_delay){Parameter1='ARETI_Rete_5', Parameter2=1, Parameter3='Iside', resources=|, Parameter10=off, codeupdate=off, step_received=|, step_computed=, dynamic_computed=, step_sended=|, id_entity=476, id_project=14, id_type=82, name_type=Reti_Sito, color=#45B5ED}
      mask resources=|
      | *** INPUT RESOURCES ***
      | NUM_INPUTS 3
      | CYBER_FAULT (25)
      | Reti_QoS (2)
      | NODO_CYBER_QoS (2)
      |
      | *** STATE VARIABLES ***
      | NUM_VARIABLES 34
      | Operative_Level(NUMERIC)(1)(1)
      | Dos_attack(NUMERIC)(1)(0)
      | MITM_attack(NUMERIC)(1)(0)
      | Virus_Attack(NUMERIC)(1)(0)
      | Port_Scan_Attack(NUMERIC)(1)(0)
      | Cyber_Fault(NUMERIC_ARRAY)(25)(0  0  0  0  0  0  0  0  0  0  0  0  0  0  0  0  0  0  0  0  0  0  0  0  0)
      | BGP_hijacking(NUMERIC)(1)(0)
      | Mechanical_Fault(NUMERIC)(1)(0)
      | Unauthorized_Access(NUMERIC)(1)(0)
      | Conn_Fault(NUMERIC)(1)(0)
      | BotNet_Attack(NUMERIC)(1)(0)
      | Data_Corruption(NUMERIC)(1)(0)
      | Rouge_Access(NUMERIC)(1)(0)
      | syslog_adm_login(NUMERIC)(1)(0)
      | SW_Change(NUMERIC)(1)(0)
      | Config_Change(NUMERIC)(1)(0)
      | Port_Saturation(NUMERIC)(1)(0)
      | Congestion_Fault(NUMERIC)(1)(0)
      | Physical_Fault(NUMERIC)(1)(0)
      | Route2(NUMERIC)(1)(0)
      | Route_Poisoning(NUMERIC)(1)(0)
      | Interface_Down(NUMERIC)(1)(0)
      | Port_Isolation(NUMERIC)(1)(0)
      | Unknown_Device(NUMERIC)(1)(0)
      | USB_Device_Insertion(NUMERIC)(1)(0)
      | Risorsa(NUMERIC)(1)(0)
      | GEO_localization(STRING)(100)()
      | SW_Fault(NUMERIC)(1)(0)
      | Internal_Cyber_Risk(NUMERIC)(1)(0)
      | Data_Breach(NUMERIC)(1)(0)
      | Ransomware(NUMERIC)(1)(0)
      | Op_Level2(NUMERIC_ARRAY)(2)(0  0)
      | Possibility_Value(NUMERIC)(1)(0)
      | Necessity_Value(NUMERIC)(1)(0)
      |
      | *** OUTPUT RESOURCES ***
      | NUM_OUTPUTS 2
      | CYBER_FAULT (25)
      | Reti_QoS (2)
      mask step_received=|
      | cyber_event=zeros(1,25);
      | cyber_event(1)=Dos_attack;
      | cyber_event(2)=MITM_attack;
      | cyber_event(3)=Virus_Attack;
      | cyber_event(4)=Port_Scan_Attack;
      | cyber_event(5)=BGP_hijacking;
      | cyber_event(6)=BotNet_Attack;
      | cyber_event(7)=Data_Corruption;
      | cyber_event(8)=SW_Change;
      | cyber_event(9)=Config_Change;
      | cyber_event(10)=Port_Saturation;
      | cyber_event(11)=Data_Breach;
      | cyber_event(12)=Unauthorized_Access;
      | cyber_event(13)=Unknown_Device;
      | cyber_event(14)=Congestion_Fault;
      | cyber_event(15)=Interface_Down;
      | cyber_event(16)=Port_Isolation;
      | cyber_event(17)=Rouge_Access;
      | cyber_event(18)=Route_Poisoning;
      | cyber_event(19)=SW_Fault;
      | cyber_event(20)=syslog_adm_login;
      | cyber_event(21)=USB_Device_Insertion;
      | cyber_event(22)=Ransomware;
      | cyber_event(23)=0;
      | cyber_event(24)=0;
      | cyber_event(25)=0;
      |
      | Cyber_Fault=max(CYBER_FAULT, transpose(cyber_event));
      |
      | Conn_Fault=max([Dos_attack BGP_hijacking Route_Poisoning Interface_Down Mechanical_Fault] );
      |
      | Operative_Level=min([(1-Conn_Fault) (1-0.5*max(Cyber_Fault))  mean(Reti_QoS)  mean(NODO_CYBER_QoS)]);
      |
      | % Il primo elemento rappersenta possibility e si combima
      | % con il max in quanto rende conto del caso migliore
      | % (perche OL)
      |
      | Op_Level2(1)=  min([1-0.3*max(Cyber_Fault) max([use_elem(Reti_QoS,1) use_elem(NODO_CYBER_QoS,1)]) 1-Conn_Fault]);
      |
      | % Il secondo elemento rappersenta necessity e si combima
      | % con il min in quanto rende conto del caso peggiore
      | % (perche OL)
      |
      | Op_Level2(2)= min([1-0.6*max(Cyber_Fault) min([use_elem(Reti_QoS,2) use_elem(NODO_CYBER_QoS,2)]) 1-Conn_Fault]);
      |
      | Possibility_Value = Op_Level2(1);
      | Necessity_Value = Op_Level2(2);
      mask step_sended=|
      | CYBER_FAULT=Cyber_Fault;
      |
      |
      | Reti_QoS=Op_Level2;
      mask prompts: Parameter1 "entity name"; Parameter2 "sampling time"; Parameter3 "project"; resources "input resources and state variables"; Parameter10 "Bring state variables to output"; codeupdate "update code from mask"
      mask help: This is a level-2 MATLAB file S-function which demonstrates CISIA entity
      mask DialogControl Container1 Prompt: All parameters
      mask Display: disp('Reti_Sito')
  ARETI_Serv_Informatico_1 (469) : M-S-Function  FunctionName=cisia_msfun  Parameters=Parameter1, Parameter2, Parameter3, resources, Parameter10, codeupdate, step_received, step_computed, dynamic_computed, step_sended, id_entity, id_project, id_type, name_type, color  mask(S-function:msfcn_unit_delay){Parameter1='ARETI_Serv_Informatico_1', Parameter2=1, Parameter3='Iside', resources=|, Parameter10=off, codeupdate=off, step_received=|, step_computed=, dynamic_computed=, step_sended=|, id_entity=469, id_project=14, id_type=83, name_type=Servizi_Informatici, color=#6FD0E8}
      mask resources=|
      | *** INPUT RESOURCES ***
      | NUM_INPUTS 6
      | CYBER_FAULT (25)
      | Sistemi_Informativi_QoS (2)
      | Reti_QoS (2)
      | Servizi_Informatici_QoS (2)
      | BENE_ICT_QoS (2)
      | EXT_SERVICE (1)
      |
      | *** STATE VARIABLES ***
      | NUM_VARIABLES 31
      | Operative_Level(NUMERIC)(1)(1)
      | Dos_attack(NUMERIC)(1)(0)
      | MITM_attack(NUMERIC)(1)(0)
      | Virus_Attack(NUMERIC)(1)(0)
      | Port_Scan_Attack(NUMERIC)(1)(0)
      | Cyber_Fault(NUMERIC_ARRAY)(25)(0  0  0  0  0  0  0  0  0  0  0  0  0  0  0  0  0  0  0  0  0  0  0  0  0)
      | BGP_hijacking(NUMERIC)(1)(0)
      | Mechanical_Fault(NUMERIC)(1)(0)
      | Unauthorized_Access(NUMERIC)(1)(0)
      | Service_Fault(NUMERIC)(1)(0)
      | BotNet_Attack(NUMERIC)(1)(0)
      | Data_Corruption(NUMERIC)(1)(0)
      | Rouge_Access(NUMERIC)(1)(0)
      | syslog_adm_login(NUMERIC)(1)(0)
      | SW_Change(NUMERIC)(1)(0)
      | Config_Change(NUMERIC)(1)(0)
      | Port_Saturation(NUMERIC)(1)(0)
      | Congestion_Fault(NUMERIC)(1)(0)
      | Route2(NUMERIC)(1)(0)
      | Route_Poisoning(NUMERIC)(1)(0)
      | Interface_Down(NUMERIC)(1)(0)
      | Port_Isolation(NUMERIC)(1)(0)
      | Unknown_Device(NUMERIC)(1)(0)
      | USB_Device_Insertion(NUMERIC)(1)(0)
      | SW_Fault(NUMERIC)(1)(0)
      | Internal_Cyber_Risk(NUMERIC)(1)(0)
      | Data_Breach(NUMERIC)(1)(0)
      | Ransomware(NUMERIC)(1)(0)
      | Op_Level2(NUMERIC_ARRAY)(2)(0  0)
      | Possibility_Value(NUMERIC)(1)(0)
      | Necessity_Value(NUMERIC)(1)(0)
      |
      | *** OUTPUT RESOURCES ***
      | NUM_OUTPUTS 2
      | CYBER_FAULT (25)
      | Servizi_Informatici_QoS (2)
      mask step_received=|
      | cyber_event=zeros(1,25);
      | cyber_event(1)=Dos_attack;
      | cyber_event(2)=MITM_attack;
      | cyber_event(3)=Virus_Attack;
      | cyber_event(4)=Port_Scan_Attack;
      | cyber_event(5)=BGP_hijacking;
      | cyber_event(6)=BotNet_Attack;
      | cyber_event(7)=Data_Corruption;
      | cyber_event(8)=SW_Change;
      | cyber_event(9)=Config_Change;
      | cyber_event(10)=Port_Saturation;
      | cyber_event(11)=Data_Breach;
      | cyber_event(12)=Unauthorized_Access;
      | cyber_event(13)=Unknown_Device;
      | cyber_event(14)=Congestion_Fault;
      | cyber_event(15)=Interface_Down;
      | cyber_event(16)=Port_Isolation;
      | cyber_event(17)=Rouge_Access;
      | cyber_event(18)=Route_Poisoning;
      | cyber_event(19)=SW_Fault;
      | cyber_event(20)=syslog_adm_login;
      | cyber_event(21)=USB_Device_Insertion;
      | cyber_event(22)=Ransomware;
      | cyber_event(23)=0;
      | cyber_event(24)=0;
      | cyber_event(25)=0;
      |
      | Cyber_Fault=max(CYBER_FAULT, transpose(cyber_event));
      |
      | SW_Fault=max([Virus_Attack Data_Corruption SW_Change] );
      |
      | Service_Fault=1-EXT_SERVICE;
      |
      | Operative_Level=min([(1-Service_Fault) (1-SW_Fault) (1- 0.5 * max(Cyber_Fault))  mean(Reti_QoS)  mean(Sistemi_Informativi_QoS) mean(Servizi_Informatici_QoS)  mean(BENE_ICT_QoS)]);
      |
      | % Il primo elemento rappersenta possibility e si combima
      | % con il max in quanto rende conto del caso migliore
      | % (perche OL)
      |
      | Op_Level2(1)=  min([1-0.3*max(Cyber_Fault) max([use_elem(Reti_QoS,1) use_elem(Sistemi_Informativi_QoS,1) use_elem(Servizi_Informatici_QoS,1) use_elem(BENE_ICT_QoS,1)]) 1-Service_Fault (1-SW_Fault)]);
      |
      | % Il secondo elemento rappersenta necessity e si combima
      | % con il min in quanto rende conto del caso peggiore
      | % (perche OL)
      |
      | Op_Level2(2)= min([1-0.6*max(Cyber_Fault) min([use_elem(Reti_QoS,2) use_elem(Sistemi_Informativi_QoS,2) use_elem(Servizi_Informatici_QoS,2) use_elem(BENE_ICT_QoS,2)]) 1-Service_Fault 1-SW_Fault]);
      |
      | Possibility_Value = Op_Level2(1);
      | Necessity_Value = Op_Level2(2);
      mask step_sended=|
      | CYBER_FAULT=Cyber_Fault;
      |
      | Servizi_Informatici_QoS=Op_Level2;
      mask prompts: Parameter1 "entity name"; Parameter2 "sampling time"; Parameter3 "project"; resources "input resources and state variables"; Parameter10 "Bring state variables to output"; codeupdate "update code from mask"
      mask help: This is a level-2 MATLAB file S-function which demonstrates CISIA entity
      mask DialogControl Container1 Prompt: All parameters
      mask Display: disp('Servizi_Informatici');port_label('input',4,'\color{yellow}\spadesuit','texmode','on');port_label('input',5,'\color{yellow}\spadesuit','texmode','on')
  ARETI_Sist_Informativo_1 (470) : M-S-Function  FunctionName=cisia_msfun  Parameters=Parameter1, Parameter2, Parameter3, resources, Parameter10, codeupdate, step_received, step_computed, dynamic_computed, step_sended, id_entity, id_project, id_type, name_type, color  mask(S-function:msfcn_unit_delay){Parameter1='ARETI_Sist_Informativo_1', Parameter2=1, Parameter3='Iside', resources=|, Parameter10=off, codeupdate=off, step_received=|, step_computed=, dynamic_computed=, step_sended=|, id_entity=470, id_project=14, id_type=81, name_type=Sistemi_Informativi, color=#59F2F7}
      mask resources=|
      | *** INPUT RESOURCES ***
      | NUM_INPUTS 5
      | CYBER_FAULT (25)
      | Sistemi_Informativi_QoS (2)
      | Reti_QoS (2)
      | Servizi_Informatici_QoS (2)
      | EXT_SERVICE (1)
      |
      | *** STATE VARIABLES ***
      | NUM_VARIABLES 33
      | Operative_Level(NUMERIC)(1)(1)
      | Dos_attack(NUMERIC)(1)(0)
      | MITM_attack(NUMERIC)(1)(0)
      | Virus_Attack(NUMERIC)(1)(0)
      | Port_Scan_Attack(NUMERIC)(1)(0)
      | Cyber_Fault(NUMERIC_ARRAY)(25)(0  0  0  0  0  0  0  0  0  0  0  0  0  0  0  0  0  0  0  0  0  0  0  0  0)
      | BGP_hijacking(NUMERIC)(1)(0)
      | Mechanical_Fault(NUMERIC)(1)(0)
      | Power_Fault(NUMERIC)(1)(0)
      | Unauthorized_Access(NUMERIC)(1)(0)
      | Consumed_Services(NUMERIC_ARRAY)(10)(0  0  0  0  0  0  0  0  0  0)
      | Service_Fault(NUMERIC)(1)(0)
      | BotNet_Attack(NUMERIC)(1)(0)
      | Data_Corruption(NUMERIC)(1)(0)
      | Rouge_Access(NUMERIC)(1)(0)
      | syslog_adm_login(NUMERIC)(1)(0)
      | SW_Change(NUMERIC)(1)(0)
      | Config_Change(NUMERIC)(1)(0)
      | Port_Saturation(NUMERIC)(1)(0)
      | Congestion_Fault(NUMERIC)(1)(0)
      | Route_Poisoning(NUMERIC)(1)(0)
      | Interface_Down(NUMERIC)(1)(0)
      | Port_Isolation(NUMERIC)(1)(0)
      | Unknown_Device(NUMERIC)(1)(0)
      | USB_Device_Insertion(NUMERIC)(1)(0)
      | Computational_Fault(NUMERIC)(1)(0)
      | SW_Fault(NUMERIC)(1)(0)
      | Internal_Cyber_Risk(NUMERIC)(1)(0)
      | Data_Breach(NUMERIC)(1)(0)
      | Ransomware(NUMERIC)(1)(0)
      | Op_Level2(NUMERIC_ARRAY)(2)(0  0)
      | Possibility_Value(NUMERIC)(1)(0)
      | Necessity_Value(NUMERIC)(1)(0)
      |
      | *** OUTPUT RESOURCES ***
      | NUM_OUTPUTS 2
      | CYBER_FAULT (25)
      | Sistemi_Informativi_QoS (2)
      mask step_received=|
      | cyber_event=zeros(1,25);
      | cyber_event(1)=Dos_attack;
      | cyber_event(2)=MITM_attack;
      | cyber_event(3)=Virus_Attack;
      | cyber_event(4)=Port_Scan_Attack;
      | cyber_event(5)=BGP_hijacking;
      | cyber_event(6)=BotNet_Attack;
      | cyber_event(7)=Data_Corruption;
      | cyber_event(8)=SW_Change;
      | cyber_event(9)=Config_Change;
      | cyber_event(10)=Port_Saturation;
      | cyber_event(11)=Data_Breach;
      | cyber_event(12)=Unauthorized_Access;
      | cyber_event(13)=Unknown_Device;
      | cyber_event(14)=Congestion_Fault;
      | cyber_event(15)=Interface_Down;
      | cyber_event(16)=Port_Isolation;
      | cyber_event(17)=Rouge_Access;
      | cyber_event(18)=Route_Poisoning;
      | cyber_event(19)=SW_Fault;
      | cyber_event(20)=syslog_adm_login;
      | cyber_event(21)=USB_Device_Insertion;
      | cyber_event(22)=Ransomware;
      | cyber_event(23)=0;
      | cyber_event(24)=0;
      | cyber_event(25)=0;
      |
      | Cyber_Fault=max(CYBER_FAULT, transpose(cyber_event));
      |
      | Computational_Fault=max([Dos_attack Virus_Attack BotNet_Attack Config_Change Mechanical_Fault] );
      |
      | Service_Fault=1-EXT_SERVICE;
      |
      | Operative_Level=min([(1-Service_Fault) (1-Computational_Fault) (1-0.5*max(Cyber_Fault))  mean(Reti_QoS)  mean(Sistemi_Informativi_QoS)  mean(Servizi_Informatici_QoS)]);
      |
      | % Il primo elemento rappersenta possibility e si combima
      | % con il max in quanto rende conto del caso migliore
      | % (perche OL)
      |
      | Op_Level2(1)=  min([1-0.3*max(Cyber_Fault) max([use_elem(Reti_QoS,1) use_elem(Sistemi_Informativi_QoS,1) use_elem(Servizi_Informatici_QoS,1)]) 1-Service_Fault (1-Computational_Fault)]);
      |
      | % Il secondo elemento rappersenta necessity e si combima
      | % con il min in quanto rende conto del caso peggiore
      | % (perche OL)
      |
      | Op_Level2(2)= min([1-0.6*max(Cyber_Fault) min([use_elem(Reti_QoS,2) use_elem(Sistemi_Informativi_QoS,2) use_elem(Servizi_Informatici_QoS,2)]) 1-Service_Fault 1-Computational_Fault]);
      |
      | Possibility_Value = Op_Level2(1);
      | Necessity_Value = Op_Level2(2);
      mask step_sended=|
      | CYBER_FAULT=Cyber_Fault;
      |
      | Sistemi_Informativi_QoS=Op_Level2;
      mask prompts: Parameter1 "entity name"; Parameter2 "sampling time"; Parameter3 "project"; resources "input resources and state variables"; Parameter10 "Bring state variables to output"; codeupdate "update code from mask"
      mask help: This is a level-2 MATLAB file S-function which demonstrates CISIA entity
      mask DialogControl Container1 Prompt: All parameters
      mask Display: disp('Sistemi_Informativi');port_label('input',1,'\color{yellow}\spadesuit','texmode','on');port_label('input',2,'\color{yellow}\spadesuit','texmode','on');port_label('input',3,'\color{yellow}\spadesuit','texmode','on');port_label('input',4,'\color{yellow}\spadesuit','texmode','on')
  ARETI_Sist_Informativo_2 (471) : M-S-Function  FunctionName=cisia_msfun  Parameters=Parameter1, Parameter2, Parameter3, resources, Parameter10, codeupdate, step_received, step_computed, dynamic_computed, step_sended, id_entity, id_project, id_type, name_type, color  mask(S-function:msfcn_unit_delay){Parameter1='ARETI_Sist_Informativo_2', Parameter2=1, Parameter3='Iside', resources=|, Parameter10=off, codeupdate=off, step_received=|, step_computed=, dynamic_computed=, step_sended=|, id_entity=471, id_project=14, id_type=81, name_type=Sistemi_Informativi, color=#59F2F7}
      mask resources=|
      | *** INPUT RESOURCES ***
      | NUM_INPUTS 5
      | CYBER_FAULT (25)
      | Sistemi_Informativi_QoS (2)
      | Reti_QoS (2)
      | Servizi_Informatici_QoS (2)
      | EXT_SERVICE (1)
      |
      | *** STATE VARIABLES ***
      | NUM_VARIABLES 33
      | Operative_Level(NUMERIC)(1)(1)
      | Dos_attack(NUMERIC)(1)(0)
      | MITM_attack(NUMERIC)(1)(0)
      | Virus_Attack(NUMERIC)(1)(0)
      | Port_Scan_Attack(NUMERIC)(1)(0)
      | Cyber_Fault(NUMERIC_ARRAY)(25)(0  0  0  0  0  0  0  0  0  0  0  0  0  0  0  0  0  0  0  0  0  0  0  0  0)
      | BGP_hijacking(NUMERIC)(1)(0)
      | Mechanical_Fault(NUMERIC)(1)(0)
      | Power_Fault(NUMERIC)(1)(0)
      | Unauthorized_Access(NUMERIC)(1)(0)
      | Consumed_Services(NUMERIC_ARRAY)(10)(0  0  0  0  0  0  0  0  0  0)
      | Service_Fault(NUMERIC)(1)(0)
      | BotNet_Attack(NUMERIC)(1)(0)
      | Data_Corruption(NUMERIC)(1)(0)
      | Rouge_Access(NUMERIC)(1)(0)
      | syslog_adm_login(NUMERIC)(1)(0)
      | SW_Change(NUMERIC)(1)(0)
      | Config_Change(NUMERIC)(1)(0)
      | Port_Saturation(NUMERIC)(1)(0)
      | Congestion_Fault(NUMERIC)(1)(0)
      | Route_Poisoning(NUMERIC)(1)(0)
      | Interface_Down(NUMERIC)(1)(0)
      | Port_Isolation(NUMERIC)(1)(0)
      | Unknown_Device(NUMERIC)(1)(0)
      | USB_Device_Insertion(NUMERIC)(1)(0)
      | Computational_Fault(NUMERIC)(1)(0)
      | SW_Fault(NUMERIC)(1)(0)
      | Internal_Cyber_Risk(NUMERIC)(1)(0)
      | Data_Breach(NUMERIC)(1)(0)
      | Ransomware(NUMERIC)(1)(0)
      | Op_Level2(NUMERIC_ARRAY)(2)(0  0)
      | Possibility_Value(NUMERIC)(1)(0)
      | Necessity_Value(NUMERIC)(1)(0)
      |
      | *** OUTPUT RESOURCES ***
      | NUM_OUTPUTS 2
      | CYBER_FAULT (25)
      | Sistemi_Informativi_QoS (2)
      mask step_received=|
      | cyber_event=zeros(1,25);
      | cyber_event(1)=Dos_attack;
      | cyber_event(2)=MITM_attack;
      | cyber_event(3)=Virus_Attack;
      | cyber_event(4)=Port_Scan_Attack;
      | cyber_event(5)=BGP_hijacking;
      | cyber_event(6)=BotNet_Attack;
      | cyber_event(7)=Data_Corruption;
      | cyber_event(8)=SW_Change;
      | cyber_event(9)=Config_Change;
      | cyber_event(10)=Port_Saturation;
      | cyber_event(11)=Data_Breach;
      | cyber_event(12)=Unauthorized_Access;
      | cyber_event(13)=Unknown_Device;
      | cyber_event(14)=Congestion_Fault;
      | cyber_event(15)=Interface_Down;
      | cyber_event(16)=Port_Isolation;
      | cyber_event(17)=Rouge_Access;
      | cyber_event(18)=Route_Poisoning;
      | cyber_event(19)=SW_Fault;
      | cyber_event(20)=syslog_adm_login;
      | cyber_event(21)=USB_Device_Insertion;
      | cyber_event(22)=Ransomware;
      | cyber_event(23)=0;
      | cyber_event(24)=0;
      | cyber_event(25)=0;
      |
      | Cyber_Fault=max(CYBER_FAULT, transpose(cyber_event));
      |
      | Computational_Fault=max([Dos_attack Virus_Attack BotNet_Attack Config_Change Mechanical_Fault] );
      |
      | Service_Fault=1-EXT_SERVICE;
      |
      | Operative_Level=min([(1-Service_Fault) (1-Computational_Fault) (1-0.5*max(Cyber_Fault))  mean(Reti_QoS)  mean(Sistemi_Informativi_QoS)  mean(Servizi_Informatici_QoS)]);
      |
      | % Il primo elemento rappersenta possibility e si combima
      | % con il max in quanto rende conto del caso migliore
      | % (perche OL)
      |
      | Op_Level2(1)=  min([1-0.3*max(Cyber_Fault) max([use_elem(Reti_QoS,1) use_elem(Sistemi_Informativi_QoS,1) use_elem(Servizi_Informatici_QoS,1)]) 1-Service_Fault (1-Computational_Fault)]);
      |
      | % Il secondo elemento rappersenta necessity e si combima
      | % con il min in quanto rende conto del caso peggiore
      | % (perche OL)
      |
      | Op_Level2(2)= min([1-0.6*max(Cyber_Fault) min([use_elem(Reti_QoS,2) use_elem(Sistemi_Informativi_QoS,2) use_elem(Servizi_Informatici_QoS,2)]) 1-Service_Fault 1-Computational_Fault]);
      |
      | Possibility_Value = Op_Level2(1);
      | Necessity_Value = Op_Level2(2);
      mask step_sended=|
      | CYBER_FAULT=Cyber_Fault;
      |
      | Sistemi_Informativi_QoS=Op_Level2;
      mask prompts: Parameter1 "entity name"; Parameter2 "sampling time"; Parameter3 "project"; resources "input resources and state variables"; Parameter10 "Bring state variables to output"; codeupdate "update code from mask"
      mask help: This is a level-2 MATLAB file S-function which demonstrates CISIA entity
      mask DialogControl Container1 Prompt: All parameters
      mask Display: disp('Sistemi_Informativi');port_label('input',2,'\color{yellow}\spadesuit','texmode','on');port_label('input',3,'\color{yellow}\spadesuit','texmode','on');port_label('input',4,'\color{yellow}\spadesuit','texmode','on')
  ARETI_cabina_primaria (426) : M-S-Function  FunctionName=cisia_msfun  Parameters=Parameter1, Parameter2, Parameter3, resources, Parameter10, codeupdate, step_received, step_computed, dynamic_computed, step_sended, id_entity, id_project, id_type, name_type, color  mask(S-function:msfcn_unit_delay){Parameter1='ARETI_cabina_primaria', Parameter2=1, Parameter3='Iside', resources=|, Parameter10=off, codeupdate=off, step_received=|, step_computed=, dynamic_computed=, step_sended=|, id_entity=426, id_project=14, id_type=104, name_type=Nodo_Cabina_Primaria, color=#DCF6F7}
      mask resources=|
      | *** INPUT RESOURCES ***
      | NUM_INPUTS 0
      |
      | *** STATE VARIABLES ***
      | NUM_VARIABLES 9
      | Operative_Level(NUMERIC)(1)(1)
      | Mechanical_Fault(NUMERIC)(1)(0)
      | Power_Fault(NUMERIC)(1)(0)
      | Flooding_Fault(NUMERIC)(1)(0)
      | Fire_Fault(NUMERIC)(1)(0)
      | Physical_Fault(NUMERIC)(1)(0)
      | Op_Level2(NUMERIC_ARRAY)(2)(0  0)
      | Possibility_Value(NUMERIC)(1)(0)
      | Necessity_Value(NUMERIC)(1)(0)
      |
      | *** OUTPUT RESOURCES ***
      | NUM_OUTPUTS 3
      | POWER (1)
      | NODO_CYBER_QoS (2)
      | NODO_PHISICAL_QoS (1)
      mask step_received=|
      | Physical_Fault = max([Mechanical_Fault Fire_Fault Flooding_Fault]);
      |
      | Operative_Level = (1-Power_Fault)*(1-Physical_Fault);
      |
      | % Il primo elemento rappersenta possibility e si combima
      | % con il max in quanto rende conto del caso migliore
      | % (perche OL)
      |
      | Op_Level2(1)=  max([1-Power_Fault 1-Physical_Fault]);
      |
      | % Il secondo elemento rappersenta necessity e si combima
      | % con il min in quanto rende conto del caso peggiore
      | % (perche OL)
      |
      | Op_Level2(2)= min([1-Power_Fault 1-Physical_Fault]);
      |
      | Possibility_Value = Op_Level2(1);
      | Necessity_Value = Op_Level2(2);
      mask step_sended=|
      | POWER = Operative_Level;
      | NODO_CYBER_QoS=Op_Level2;
      | NODO_PHISICAL_QoS=Operative_Level;
      mask prompts: Parameter1 "entity name"; Parameter2 "sampling time"; Parameter3 "project"; resources "input resources and state variables"; Parameter10 "Bring state variables to output"; codeupdate "update code from mask"
      mask help: This is a level-2 MATLAB file S-function which demonstrates CISIA entity
      mask DialogControl Container1 Prompt: All parameters
      mask Display: disp('Nodo_Cabina_Primaria')
  ARETI_cabina_secondaria (439) : M-S-Function  FunctionName=cisia_msfun  Parameters=Parameter1, Parameter2, Parameter3, resources, Parameter10, codeupdate, step_received, step_computed, dynamic_computed, step_sended, id_entity, id_project, id_type, name_type, color  mask(S-function:msfcn_unit_delay){Parameter1='ARETI_cabina_secondaria', Parameter2=1, Parameter3='Iside', resources=|, Parameter10=off, codeupdate=off, step_received=|, step_computed=, dynamic_computed=, step_sended=|, id_entity=439, id_project=14, id_type=107, name_type=Nodo_Cabina_Secondaria, color=#DCF6F7}
      mask resources=|
      | *** INPUT RESOURCES ***
      | NUM_INPUTS 1
      | POWER (1)
      |
      | *** STATE VARIABLES ***
      | NUM_VARIABLES 9
      | Operative_Level(NUMERIC)(1)(1)
      | Mechanical_Fault(NUMERIC)(1)(0)
      | Power_Fault(NUMERIC)(1)(0)
      | Flooding_Fault(NUMERIC)(1)(0)
      | Fire_Fault(NUMERIC)(1)(0)
      | Physical_Fault(NUMERIC)(1)(0)
      | Op_Level2(NUMERIC_ARRAY)(2)(0  0)
      | Possibility_Value(NUMERIC)(1)(0)
      | Necessity_Value(NUMERIC)(1)(0)
      |
      | *** OUTPUT RESOURCES ***
      | NUM_OUTPUTS 3
      | POWER (1)
      | NODO_CYBER_QoS (2)
      | NODO_PHISICAL_QoS (1)
      mask step_received=|
      | Power_Fault = 1-POWER;
      | Physical_Fault = max([Mechanical_Fault Fire_Fault Flooding_Fault]);
      |
      | Operative_Level = (1-Power_Fault)*(1-Physical_Fault);
      |
      | % Il primo elemento rappersenta possibility e si combima
      | % con il max in quanto rende conto del caso migliore
      | % (perche OL)
      |
      | Op_Level2(1)=  max([1-Power_Fault 1-Physical_Fault]);
      |
      | % Il secondo elemento rappersenta necessity e si combima
      | % con il min in quanto rende conto del caso peggiore
      | % (perche OL)
      |
      | Op_Level2(2)= min([1-Power_Fault 1-Physical_Fault]);
      |
      | Possibility_Value = Op_Level2(1);
      | Necessity_Value = Op_Level2(2);
      mask step_sended=|
      | POWER = Operative_Level;
      | NODO_CYBER_QoS=Op_Level2;
      | NODO_PHISICAL_QoS=Operative_Level;
      mask prompts: Parameter1 "entity name"; Parameter2 "sampling time"; Parameter3 "project"; resources "input resources and state variables"; Parameter10 "Bring state variables to output"; codeupdate "update code from mask"
      mask help: This is a level-2 MATLAB file S-function which demonstrates CISIA entity
      mask DialogControl Container1 Prompt: All parameters
      mask Display: disp('Nodo_Cabina_Secondaria')
  ELE2_org (544) : M-S-Function  FunctionName=cisia_msfun  Parameters=Parameter1, Parameter2, Parameter3, resources, Parameter10, codeupdate, step_received, step_computed, dynamic_computed, step_sended, id_entity, id_project, id_type, name_type, color  mask(S-function:msfcn_unit_delay){Parameter1='ELE2_org', Parameter2=1, Parameter3='Iside', resources=|, Parameter10=off, codeupdate=off, step_received=|, step_computed=, dynamic_computed=, step_sended=|, id_entity=544, id_project=14, id_type=118, name_type=Organization, color=#A2142F}
      mask resources=|
      | *** INPUT RESOURCES ***
      | NUM_INPUTS 6
      | CYBER_FAULT (25)
      | BENE_ICT_QoS (2)
      | FUNZIONI_ESSENZIALI (10)
      | SERVIZI_ESSENZIALI (10)
      | CYBER_RISK (3)
      | PHYSICAL_STRENGTH (1)
      |
      | *** STATE VARIABLES ***
      | NUM_VARIABLES 35
      | Operative_Level(NUMERIC)(1)(1)
      | Dos_attack(NUMERIC)(1)(0)
      | MITM_attack(NUMERIC)(1)(0)
      | Virus_Attack(NUMERIC)(1)(0)
      | Port_Scan_Attack(NUMERIC)(1)(0)
      | Cyber_Fault(NUMERIC_ARRAY)(25)(0  0  0  0  0  0  0  0  0  0  0  0  0  0  0  0  0  0  0  0  0  0  0  0  0)
      | BGP_hijacking(NUMERIC)(1)(0)
      | Mechanical_Fault(NUMERIC)(1)(0)
      | Unauthorized_Access(NUMERIC)(1)(0)
      | Conn_Fault(NUMERIC)(1)(0)
      | BotNet_Attack(NUMERIC)(1)(0)
      | Data_Corruption(NUMERIC)(1)(0)
      | Rouge_Access(NUMERIC)(1)(0)
      | syslog_adm_login(NUMERIC)(1)(0)
      | SW_Change(NUMERIC)(1)(0)
      | Config_Change(NUMERIC)(1)(0)
      | Port_Saturation(NUMERIC)(1)(0)
      | Congestion_Fault(NUMERIC)(1)(0)
      | Physical_Fault(NUMERIC)(1)(0)
      | Route_Poisoning(NUMERIC)(1)(0)
      | Interface_Down(NUMERIC)(1)(0)
      | Port_Isolation(NUMERIC)(1)(0)
      | Unknown_Device(NUMERIC)(1)(0)
      | USB_Device_Insertion(NUMERIC)(1)(0)
      | SW_Fault(NUMERIC)(1)(0)
      | Servizi_Essenziali(NUMERIC_ARRAY)(10)(0  0  0  0  0  0  0  0  0  0)
      | Funzioni_Essenziali(NUMERIC_ARRAY)(10)(0  0  0  0  0  0  0  0  0  0)
      | Internal_Cyber_Risk(NUMERIC)(1)(0)
      | Data_Breach(NUMERIC)(1)(0)
      | availability_fault(NUMERIC)(1)(0)
      | Ransomware(NUMERIC)(1)(0)
      | ExternalCyberFault(NUMERIC_ARRAY)(3)(0  0  0)
      | Op_Level2(NUMERIC_ARRAY)(2)(1  1)
      | Possibility_Value(NUMERIC)(1)(0)
      | Necessity_Value(NUMERIC)(1)(0)
      |
      | *** OUTPUT RESOURCES ***
      | NUM_OUTPUTS 6
      | CYBER_FAULT (25)
      | FUNZIONI_ESSENZIALI (10)
      | SERVIZI_ESSENZIALI (10)
      | CYBER_RISK (3)
      | ORG_QoS (2)
      | EXTERNAL_CYBER_IMPACT (1)
      mask step_received=|
      | cyber_event=zeros(1,25);
      | cyber_event(1)=Dos_attack;
      | cyber_event(2)=MITM_attack;
      | cyber_event(3)=Virus_Attack;
      | cyber_event(4)=Port_Scan_Attack;
      | cyber_event(5)=BGP_hijacking;
      | cyber_event(6)=BotNet_Attack;
      | cyber_event(7)=Data_Corruption;
      | cyber_event(8)=SW_Change;
      | cyber_event(9)=Config_Change;
      | cyber_event(10)=Port_Saturation;
      | cyber_event(11)=Data_Breach;
      | cyber_event(12)=Unauthorized_Access;
      | cyber_event(13)=Unknown_Device;
      | cyber_event(14)=Congestion_Fault;
      | cyber_event(15)=Interface_Down;
      | cyber_event(16)=Port_Isolation;
      | cyber_event(17)=Rouge_Access;
      | cyber_event(18)=Route_Poisoning;
      | cyber_event(19)=SW_Fault;
      | cyber_event(20)=syslog_adm_login;
      | cyber_event(21)=USB_Device_Insertion;
      | cyber_event(22)=Ransomware;
      | cyber_event(23)=0;
      | cyber_event(24)=0;
      | cyber_event(25)=0;
      |
      | Cyber_Fault=max(CYBER_FAULT, transpose(cyber_event));
      |
      |
      | Conn_Fault=max([Dos_attack BGP_hijacking Route_Poisoning Interface_Down Mechanical_Fault] );
      |
      |
      | Servizi_Essenziali=SERVIZI_ESSENZIALI;
      | Funzioni_Essenziali=FUNZIONI_ESSENZIALI;
      |
      | ExternalCyberFault=CYBER_RISK;
      |
      | Operative_Level=min([1-0.5*max(Cyber_Fault) mean(BENE_ICT_QoS) PHYSICAL_STRENGTH]);
      |
      |
      | Physical_Fault=1-PHYSICAL_STRENGTH;
      |
      | % Il primo elemento rappersenta possibility e si combima
      | % con il max in quanto rende conto del caso migliore
      | % (perche OL)
      |
      | Op_Level2(1)=  min([1-0.3*max(Cyber_Fault) BENE_ICT_QoS(1) PHYSICAL_STRENGTH]);
      |
      | % Il secondo elemento rappersenta necessity e si combima
      | % con il min in quanto rende conto del caso peggiore
      | % (perche OL)
      |
      | Op_Level2(2)= min([1-0.6*max(Cyber_Fault) BENE_ICT_QoS(2) PHYSICAL_STRENGTH]);
      |
      | Possibility_Value = Op_Level2(1);
      | Necessity_Value = Op_Level2(2);
      mask step_sended=|
      | SERVIZI_ESSENZIALI=Servizi_Essenziali*(1-Physical_Fault);
      | FUNZIONI_ESSENZIALI=Funzioni_Essenziali*(1-Physical_Fault);
      |
      |
      | ORG_QoS = Op_Level2;
      |
      | % Need to evaluate C-I-A from Cyber_Fault
      | integrity_fault=max([Cyber_Fault(7)  Cyber_Fault(8) Cyber_Fault(22)]);
      |
      | confidentiality_fault=max([Cyber_Fault(2)  Cyber_Fault(3)  Cyber_Fault(6)  Cyber_Fault(9) Cyber_Fault(22)]);
      |
      | availability_fault=max(Cyber_Fault);
      |
      |
      | % C-I-A
      | CYBER_RISK(1)=confidentiality_fault;
      | CYBER_RISK(2)=integrity_fault;
      | CYBER_RISK(3)=availability_fault;
      |
      | % Need to filter the propagable ones
      | CYBER_FAULT = Cyber_Fault;
      |
      |
      | % Need to map from external risks to internal ones
      | EXTERNAL_CYBER_IMPACT=max(ExternalCyberFault);
      mask prompts: Parameter1 "entity name"; Parameter2 "sampling time"; Parameter3 "project"; resources "input resources and state variables"; Parameter10 "Bring state variables to output"; codeupdate "update code from mask"
      mask help: This is a level-2 MATLAB file S-function which demonstrates CISIA entity
      mask DialogControl Container1 Prompt: All parameters
      mask Display: disp('Organization')
  MinMax{2,5..7} (4 alike) : MinMax  Function=max  Inputs=2
  MinMax3 : MinMax  Function=max  Inputs=4
  Subsystem1 : Subsystem  mask{num_serv=1, operation1=All services required, operation2=All providers required, out_service=none, consumed1=[1 0 0 0 0 0 0 0 0 0]}
      mask prompts: num_serv "Providers in input"; operation1 "For each single service provider"; operation2 "Among providers"; out_service "Vectorial output"; consumed1 "Required 1"
      mask TypeOptions num_serv: 1
      mask TypeOptions operation1: All services required | At least one
      mask TypeOptions operation2: All providers required
      mask TypeOptions out_service: none | S1 | S2 | S3 | S4 | S5 | S6 | S7 | S8 | S9 | S10 | F1 | F2 | F3 | F4 | F5 | F6 | F7 | F8 | F9 | F10
  Subsystem2 : Subsystem  mask{num_serv=1, operation1=All services required, operation2=All providers required, out_service=S2, consumed1=[1 0 0 0 0 0 0 0 0 0]}
      mask prompts: num_serv "Providers in input"; operation1 "For each single service provider"; operation2 "Among providers"; out_service "Vectorial output"; consumed1 "Required 1"
      mask TypeOptions num_serv: 1
      mask TypeOptions operation1: All services required | At least one
      mask TypeOptions operation2: All providers required
      mask TypeOptions out_service: none | S1 | S2 | S3 | S4 | S5 | S6 | S7 | S8 | S9 | S10 | F1 | F2 | F3 | F4 | F5 | F6 | F7 | F8 | F9 | F10
  Subsystem4 : Subsystem  mask{num_serv=1, operation1=All services required, operation2=All providers required, out_service=none, consumed1=[1 0 0 0 0 0 0 0 0 0]}
      mask prompts: num_serv "Providers in input"; operation1 "For each single service provider"; operation2 "Among providers"; out_service "Vectorial output"; consumed1 "Required 1"
      mask TypeOptions num_serv: 1
      mask TypeOptions operation1: All services required | At least one
      mask TypeOptions operation2: All providers required
      mask TypeOptions out_service: none | S1 | S2 | S3 | S4 | S5 | S6 | S7 | S8 | S9 | S10 | F1 | F2 | F3 | F4 | F5 | F6 | F7 | F8 | F9 | F10
  Subsystem9 : Subsystem  mask{num_serv=1, operation1=All services required, operation2=All providers required, out_service=S1, consumed1=[1 0 0 0 0 0 0 0 0 0]}
      mask prompts: num_serv "Providers in input"; operation1 "For each single service provider"; operation2 "Among providers"; out_service "Vectorial output"; consumed1 "Required 1"
      mask TypeOptions num_serv: 1
      mask TypeOptions operation1: All services required | At least one
      mask TypeOptions operation2: All providers required
      mask TypeOptions out_service: none | S1 | S2 | S3 | S4 | S5 | S6 | S7 | S8 | S9 | S10 | F1 | F2 | F3 | F4 | F5 | F6 | F7 | F8 | F9 | F10
  delay : Subsystem  mask{delay=0.9, output=ones(1,10)}
  delay1 : Subsystem  mask{delay=0.9, output=ones(1,10)}
  maxmin1 : MATLAB Function  TreatAsAtomicUnit=on
  maxmin2 : MATLAB Function  TreatAsAtomicUnit=on
  CYBER_FAULT_ELE2 : Outport
  FUNZIONI_ELE2 : Outport  Port=2
  SERVIZI_ELE2 : Outport  Port=3
  CYBER_RISK_ELE2 : Outport  Port=4
  ELE2_QoS : Outport  Port=5
  EXTERNAL_CYBER_IMPACT : Outport  Port=6
  wires:
  ELE2_org (544)/1 -> CYBER_FAULT_ELE2/1  "CYBER_FAULT"
  ELE2_org (544)/3 -> delay1/1(in)  "SERVIZI_ESSENZIALI"
  MinMax7/1 -> ELE2_org (544)/1  "CYBER_FAULT"
  maxmin2/1(y) -> ELE2_org (544)/2  "BENE_ICT_QoS"
  MinMax3/1 -> ARETI_Rete_5 (476)/1  "CYBER_FAULT"
  ARETI_BeneICT_1 (467)/1 -> MinMax7/1  "CYBER_FAULT"
  ARETI_BeneICT_1 (467)/3 -> MinMax6/1  "FUNZIONI_ESSENZIALI"
  ARETI_BeneICT_2 (468)/1 -> MinMax7/2  "CYBER_FAULT"
  ARETI_BeneICT_1 (467)/2 -> maxmin2/2(u2)  "BENE_ICT_QoS"
  ARETI_Rete_4 (475)/1 -> MinMax3/3  "CYBER_FAULT"
  MinMax6/1 -> ELE2_org (544)/3  "FUNZIONI_ESSENZIALI"
  ARETI_BeneICT_2 (468)/3 -> MinMax6/2  "FUNZIONI_ESSENZIALI"
  ARETI_Rete_3 (474)/1 -> MinMax3/2  "CYBER_FAULT"
  ARETI_Sist_Informativo_2 (471)/1 -> MinMax2/1  "CYBER_FAULT"
  ARETI_Rete_5 (476)/1 -> MinMax2/2  "CYBER_FAULT"
  ARETI_Serv_Informatico_1 (469)/1 -> ARETI_BeneICT_2 (468)/1, ARETI_BeneICT_1 (467)/1  "CYBER_FAULT"
  ARETI_BeneICT_2 (468)/2 -> maxmin2/1(u1)  "BENE_ICT_QoS"
  ARETI_Physical/1(Physical) -> ELE2_org (544)/6  "PHYSICAL_STRENGTH"
  ARETI_Sist_Informativo_1 (470)/1 -> ARETI_Sist_Informativo_2 (471)/1  "CYBER_FAULT"
  ARETI_Rete_2 (473)/1 -> MinMax3/1  "CYBER_FAULT"
  ARETI_Rete_1 (472)/1 -> ARETI_Rete_2 (473)/1  "CYBER_FAULT"
  ARETI_cabina_primaria (426)/2 -> ARETI_Rete_1 (472)/3  "NODO_CYBER_QoS"
  ARETI_cabina_primaria (426)/1 -> ARETI_cabina_secondaria (439)/1  "POWER"
  ARETI_cabina_secondaria (439)/1 -> ARETI_1_trasformatore (427)/1, ARETI_2_trasformatore (428)/1  "POWER"
  ARETI_cabina_secondaria (439)/2 -> ARETI_Rete_3 (474)/3  "NODO_CYBER_QoS"
  ARETI_1_trasformatore (427)/2 -> ARETI_Rete_4 (475)/3  "NODO_CYBER_QoS"
  ARETI_2_trasformatore (428)/2 -> ARETI_Rete_2 (473)/3  "NODO_CYBER_QoS"
  ARETI_2_trasformatore (428)/3 -> ARETI_Physical/1(N1)  "NODO_PHISICAL_QoS"
  ARETI_1_trasformatore (427)/3 -> ARETI_Physical/2(N2)  "NODO_PHISICAL_QoS"
  ARETI_cabina_secondaria (439)/3 -> ARETI_Physical/3(N3)  "NODO_PHISICAL_QoS"
  ARETI_cabina_primaria (426)/3 -> ARETI_Physical/4(N4)  "NODO_PHISICAL_QoS"
  SERVIZI_TELCO2/1 -> [SERVIZI_TELCO2]
  CYBER_RSK_TELCO2/1 -> [CYBER_RISK]
  ARETI_Rete_1 (472)/2 -> ARETI_Rete_2 (473)/2  "Reti_QoS"
  ARETI_Nodo_1 (477)/2 -> ARETI_Rete_5 (476)/3  "NODO_CYBER_QoS"
  ARETI_Nodo_1 (477)/1 -> MinMax3/4  "CYBER_FAULT"
  ARETI_Rete_2 (473)/2 -> maxmin1/1(u1)  "Reti_QoS"
  ARETI_Rete_3 (474)/2 -> maxmin1/2(u2)  "Reti_QoS"
  ARETI_Rete_4 (475)/2 -> maxmin1/3(u3)  "Reti_QoS"
  maxmin1/1(y) -> ARETI_Rete_5 (476)/2  "Reti_QoS"
  [SERVIZI_TELCO2] -> Subsystem1/1(servizio)
  Subsystem1/1(EXT) -> ARETI_Sist_Informativo_1 (470)/5, ARETI_Sist_Informativo_2 (471)/5  "EXT_SERVICE"
  ARETI_Sist_Informativo_2 (471)/2 -> ARETI_Serv_Informatico_1 (469)/2  "Sistemi_Informativi_QoS"
  MinMax2/1 -> ARETI_Serv_Informatico_1 (469)/1  "CYBER_FAULT"
  ARETI_Rete_5 (476)/2 -> ARETI_Serv_Informatico_1 (469)/3  "Reti_QoS"
  Subsystem4/1(EXT) -> ARETI_Serv_Informatico_1 (469)/6  "EXT_SERVICE"
  [SERVIZI_TELCO2] -> Subsystem4/1(servizio)
  [SERVIZI_TELCO2] -> Subsystem9/1(servizio)
  Subsystem9/2(EXT_V) -> ARETI_BeneICT_1 (467)/6  "SERVIZIO_ESTERNO"
  [SERVIZI_TELCO2] -> Subsystem2/1(servizio)
  Subsystem2/2(EXT_V) -> ARETI_BeneICT_2 (468)/6  "SERVIZIO_ESTERNO"
  MinMax5/1 -> ELE2_org (544)/4  "SERVIZI_ESSENZIALI"
  ARETI_BeneICT_1 (467)/4 -> MinMax5/1  "SERVIZI_ESSENZIALI"
  ARETI_BeneICT_2 (468)/4 -> MinMax5/2  "SERVIZI_ESSENZIALI"
  [CYBER_RISK] -> ELE2_org (544)/5  "CYBER_RISK"
  delay/1(out) -> FUNZIONI_ELE2/1
  ELE2_org (544)/2 -> delay/1(in)  "FUNZIONI_ESSENZIALI"
  ARETI_Serv_Informatico_1 (469)/2 -> ARETI_BeneICT_2 (468)/4, ARETI_BeneICT_1 (467)/4  "Servizi_Informatici_QoS"
  delay1/1(out) -> SERVIZI_ELE2/1
  ELE2_org (544)/4 -> CYBER_RISK_ELE2/1  "CYBER_RISK"
  ELE2_org (544)/5 -> ELE2_QoS/1  "ORG_QoS"
  ELE2_org (544)/6 -> EXTERNAL_CYBER_IMPACT/1  "EXTERNAL_CYBER_IMPACT"
